simulink model "ext_mode_intro"  (R2017b)
settings: Solver=FixedStepDiscrete  StartTime=0.0  StopTime=inf  FixedStep=1/100  RelTol=1e-3  EnableMultiTasking=on
InitFcn:
  | GainTune = 1;
  | alignTime = floor(398.001 * Ts);
  | EAS2TAS = 1;
  | LatDegInit = 1;
  | LngDegInit = 1;
  | msecVelDelay = 300;
  | msecPosDelay = 300;
  | msecHgtDelay = 420;
  | msecMagDelay = 30;
  | msecTasDelay = 200;
libraries: simulink x9, pixhawk_slib_sensors_actuators x3, simulink_need_slupdate x2
(part 2 of 4)

== matlab function ext_mode_intro/EKF/EKF/Subsystem/Predict Covariance ==
  data: deltaAngle input; deltaVelocity input; nextP output; states input; P input; dtIMU input; onGround input; useAirspeed input; useCompass input
%#codegen
function nextP  = CovariancePrediction(deltaAngle, ...
    deltaVelocity, ...
    states,...
    P, ...  % Previous state covariance matrix
    dtIMU, ... % IMU and prediction time step
    onGround, ... % Boolean to indicate when on ground
    useAirspeed, ... % Boolean to indicate that airspeed sensing is being used
    useCompass) % Boolean to indicate that a magnetometer is being used

dtCovPred = 0.0; % time between covariance prediction updates

persistent storedDelAng;
if isempty(storedDelAng)
    storedDelAng = single([0;0;0]);
end
persistent storedDelVel;
if isempty(storedDelVel)
    storedDelVel = single([0;0;0]);
end
persistent dt;
if isempty(dt)
    dt = single(0.0);
end
persistent skipCount;
if isempty(skipCount)
    skipCount = 0;
end

storedDelAng = storedDelAng + deltaAngle;
storedDelVel = storedDelVel + deltaVelocity;
dt = dt + dtIMU;

if dt >= dtCovPred
    
    % Set the filter process noise - this consists of a very small amount to
    % cover processing errors. IMU errors are already built into the
    % equations
    % It  includes the process noise required for evolution of the IMU bias
    % errors, wind velocity and magnetic field states
    
    windVelSigma  = single(dt*0.1); % 0.1 m/s/s
    dAngBiasSigma = single(dt*0.05/3600*pi/180);
    dVelBiasSigma = single(dt*0.01/60);
    magEarthSigma = single(dt*10/60); % 10 mgauss per minute
    magBodySigma  = single(dt*100/60); % 100 mgauss per minute - allow to adapt more rapidly due to changes in airframe
    
    processNoise = [1e-9*ones(1,10), dAngBiasSigma*[1 1 1], dVelBiasSigma*[1 1 1], windVelSigma*[1 1], magEarthSigma*[1 1 1], magBodySigma*[1 1 1]].^2;
    
    % Specify the estimated errors on the delta angles and delta velocities
    daxCov = (dt*25.0/60*pi/180)^2;
    dayCov = (dt*25.0/60*pi/180)^2;
    dazCov = (dt*25.0/60*pi/180)^2;
    dvxCov = (dt*0.5)^2;
    dvyCov = (dt*0.5)^2;
    dvzCov = (dt*0.5)^2;
    
    dvx = deltaVelocity(1);
    dvy = deltaVelocity(2);
    dvz = deltaVelocity(3);
    dax = deltaAngle(1);
    day = deltaAngle(2);
    daz = deltaAngle(3);
    
    q0 = states(1);
    q1 = states(2);
    q2 = states(3);
    q3 = states(4);
    
    vn = states(5);
    ve = states(6);
    vd = states(7);
    
    pn = states(8);
    pe = states(9);
    pd = states(10);
    
    dax_b = states(11);
    day_b = states(12);
    daz_b = states(13);
    
    dvx_b = states(14);
    dvy_b = states(15);
    dvz_b = states(16);
    
    vwn = states(17);
    vwe = states(18);
    
    magN = states(19);
    magE = states(20);
    magD = states(21);
    
    magX = states(22);
    magY = states(23);
    magZ = states(24);
    
    % Predicted covariance
    
    SF = single(zeros(21,1));
    SF(1) = dvz - dvz_b;
    SF(2) = dvy - dvy_b;
    SF(3) = dvx - dvx_b;
    SF(4) = 2*q1*SF(3) + 2*q2*SF(2) + 2*q3*SF(1);
    SF(5) = 2*q0*SF(2) - 2*q1*SF(1) + 2*q3*SF(3);
    SF(6) = 2*q0*SF(3) + 2*q2*SF(1) - 2*q3*SF(2);
    SF(7) = day/2 - day_b/2;
    SF(8) = daz/2 - daz_b/2;
    SF(9) = dax/2 - dax_b/2;
    SF(10) = dax_b/2 - dax/2;
    SF(11) = daz_b/2 - daz/2;
    SF(12) = day_b/2 - day/2;
    SF(13) = 2*q1*SF(2);
    SF(14) = 2*q0*SF(1);
    SF(15) = q1/2;
    SF(16) = q2/2;
    SF(17) = q3/2;
    SF(18) = q3^2;
    SF(19) = q2^2;
    SF(20) = q1^2;
    SF(21) = q0^2;
    
    SG = single(zeros(8,1));
    SG(1) = q0/2;
    SG(2) = q3^2;
    SG(3) = q2^2;
    SG(4) = q1^2;
    SG(5) = q0^2;
    SG(6) = 2*q2*q3;
    SG(7) = 2*q1*q3;
    SG(8) = 2*q1*q2;
    
    SQ = single(zeros(11,1));
    SQ(1) = dvzCov*(SG(6) - 2*q0*q1)*(SG(2) - SG(3) - SG(4) + SG(5)) - dvyCov*(SG(6) + 2*q0*q1)*(SG(2) - SG(3) + SG(4) - SG(5)) + dvxCov*(SG(7) - 2*q0*q2)*(SG(8) + 2*q0*q3);
    SQ(2) = dvzCov*(SG(7) + 2*q0*q2)*(SG(2) - SG(3) - SG(4) + SG(5)) - dvxCov*(SG(7) - 2*q0*q2)*(SG(2) + SG(3) - SG(4) - SG(5)) + dvyCov*(SG(6) + 2*q0*q1)*(SG(8) - 2*q0*q3);
    SQ(3) = dvzCov*(SG(6) - 2*q0*q1)*(SG(7) + 2*q0*q2) - dvyCov*(SG(8) - 2*q0*q3)*(SG(2) - SG(3) + SG(4) - SG(5)) - dvxCov*(SG(8) + 2*q0*q3)*(SG(2) + SG(3) - SG(4) - SG(5));
    SQ(4) = (dayCov*q1*SG(1))/2 - (dazCov*q1*SG(1))/2 - (daxCov*q2*q3)/4;
    SQ(5) = (dazCov*q2*SG(1))/2 - (daxCov*q2*SG(1))/2 - (dayCov*q1*q3)/4;
    SQ(6) = (daxCov*q3*SG(1))/2 - (dayCov*q3*SG(1))/2 - (dazCov*q1*q2)/4;
    SQ(7) = (daxCov*q1*q2)/4 - (dazCov*q3*SG(1))/2 - (dayCov*q1*q2)/4;
    SQ(8) = (dazCov*q1*q3)/4 - (daxCov*q1*q3)/4 - (dayCov*q2*SG(1))/2;
    SQ(9) = (dayCov*q2*q3)/4 - (daxCov*q1*SG(1))/2 - (dazCov*q2*q3)/4;
    SQ(10) = SG(1)^2;
    SQ(11) = q1^2;
    
    SPP = single(zeros(13,1));
    SPP(1) = SF(13) + SF(14) - 2*q2*SF(3);
    SPP(2) = SF(18) - SF(19) - SF(20) + SF(21);
    SPP(3) = SF(18) - SF(19) + SF(20) - SF(21);
    SPP(4) = SF(18) + SF(19) - SF(20) - SF(21);
    SPP(5) = 2*q0*SF(3) + 2*q2*SF(1) - 2*q3*SF(2);
    SPP(6) = 2*q0*SF(2) - 2*q1*SF(1) + 2*q3*SF(3);
    SPP(7) = 2*q0*q2 - 2*q1*q3;
    SPP(8) = 2*q0*q1 - 2*q2*q3;
    SPP(9) = 2*q0*q3 - 2*q1*q2;
    SPP(10) = 2*q0*q1 + 2*q2*q3;
    SPP(11) = 2*q0*q3 + 2*q1*q2;
    SPP(12) = 2*q0*q2 + 2*q1*q3;
    SPP(13) = SF(17);
    
    nextP = single(zeros(24,24));
    nextP(1,1) = P(1,1) + P(2,1)*SF(10) + P(3,1)*SF(12) + P(4,1)*SF(11) + P(11,1)*SF(15) + P(12,1)*SF(16) + P(13,1)*SPP(13) + (daxCov*SQ(11))/4 + SF(10)*(P(1,2) + P(2,2)*SF(10) + P(3,2)*SF(12) + P(4,2)*SF(11) + P(11,2)*SF(15) + P(12,2)*SF(16) + P(13,2)*SPP(13)) + SF(12)*(P(1,3) + P(2,3)*SF(10) + P(3,3)*SF(12) + P(4,3)*SF(11) + P(11,3)*SF(15) + P(12,3)*SF(16) + P(13,3)*SPP(13)) + SF(11)*(P(1,4) + P(2,4)*SF(10) + P(3,4)*SF(12) + P(4,4)*SF(11) + P(11,4)*SF(15) + P(12,4)*SF(16) + P(13,4)*SPP(13)) + SF(15)*(P(1,11) + P(2,11)*SF(10) + P(3,11)*SF(12) + P(4,11)*SF(11) + P(11,11)*SF(15) + P(12,11)*SF(16) + P(13,11)*SPP(13)) + SF(16)*(P(1,12) + P(2,12)*SF(10) + P(3,12)*SF(12) + P(4,12)*SF(11) + P(11,12)*SF(15) + P(12,12)*SF(16) + P(13,12)*SPP(13)) + SPP(13)*(P(1,13) + P(2,13)*SF(10) + P(3,13)*SF(12) + P(4,13)*SF(11) + P(11,13)*SF(15) + P(12,13)*SF(16) + P(13,13)*SPP(13)) + (dayCov*q2^2)/4 + (dazCov*q3^2)/4;
    nextP(1,2) = P(1,2) + SQ(9) + P(2,2)*SF(10) + P(3,2)*SF(12) + P(4,2)*SF(11) + P(11,2)*SF(15) + P(12,2)*SF(16) + P(13,2)*SPP(13) + SF(9)*(P(1,1) + P(2,1)*SF(10) + P(3,1)*SF(12) + P(4,1)*SF(11) + P(11,1)*SF(15) + P(12,1)*SF(16) + P(13,1)*SPP(13)) + SF(8)*(P(1,3) + P(2,3)*SF(10) + P(3,3)*SF(12) + P(4,3)*SF(11) + P(11,3)*SF(15) + P(12,3)*SF(16) + P(13,3)*SPP(13)) + SF(12)*(P(1,4) + P(2,4)*SF(10) + P(3,4)*SF(12) + P(4,4)*SF(11) + P(11,4)*SF(15) + P(12,4)*SF(16) + P(13,4)*SPP(13)) - SF(16)*(P(1,13) + P(2,13)*SF(10) + P(3,13)*SF(12) + P(4,13)*SF(11) + P(11,13)*SF(15) + P(12,13)*SF(16) + P(13,13)*SPP(13)) + SPP(13)*(P(1,12) + P(2,12)*SF(10) + P(3,12)*SF(12) + P(4,12)*SF(11) + P(11,12)*SF(15) + P(12,12)*SF(16) + P(13,12)*SPP(13)) - (q0*(P(1,11) + P(2,11)*SF(10) + P(3,11)*SF(12) + P(4,11)*SF(11) + P(11,11)*SF(15) + P(12,11)*SF(16) + P(13,11)*SPP(13)))/2;
    nextP(1,3) = P(1,3) + SQ(8) + P(2,3)*SF(10) + P(3,3)*SF(12) + P(4,3)*SF(11) + P(11,3)*SF(15) + P(12,3)*SF(16) + P(13,3)*SPP(13) + SF(7)*(P(1,1) + P(2,1)*SF(10) + P(3,1)*SF(12) + P(4,1)*SF(11) + P(11,1)*SF(15) + P(12,1)*SF(16) + P(13,1)*SPP(13)) + SF(11)*(P(1,2) + P(2,2)*SF(10) + P(3,2)*SF(12) + P(4,2)*SF(11) + P(11,2)*SF(15) + P(12,2)*SF(16) + P(13,2)*SPP(13)) + SF(9)*(P(1,4) + P(2,4)*SF(10) + P(3,4)*SF(12) + P(4,4)*SF(11) + P(11,4)*SF(15) + P(12,4)*SF(16) + P(13,4)*SPP(13)) + SF(15)*(P(1,13) + P(2,13)*SF(10) + P(3,13)*SF(12) + P(4,13)*SF(11) + P(11,13)*SF(15) + P(12,13)*SF(16) + P(13,13)*SPP(13)) - SPP(13)*(P(1,11) + P(2,11)*SF(10) + P(3,11)*SF(12) + P(4,11)*SF(11) + P(11,11)*SF(15) + P(12,11)*SF(16) + P(13,11)*SPP(13)) - (q0*(P(1,12) + P(2,12)*SF(10) + P(3,12)*SF(12) + P(4,12)*SF(11) + P(11,12)*SF(15) + P(12,12)*SF(16) + P(13,12)*SPP(13)))/2;
    nextP(1,4) = P(1,4) + SQ(7) + P(2,4)*SF(10) + P(3,4)*SF(12) + P(4,4)*SF(11) + P(11,4)*SF(15) + P(12,4)*SF(16) + P(13,4)*SPP(13) + SF(8)*(P(1,1) + P(2,1)*SF(10) + P(3,1)*SF(12) + P(4,1)*SF(11) + P(11,1)*SF(15) + P(12,1)*SF(16) + P(13,1)*SPP(13)) + SF(7)*(P(1,2) + P(2,2)*SF(10) + P(3,2)*SF(12) + P(4,2)*SF(11) + P(11,2)*SF(15) + P(12,2)*SF(16) + P(13,2)*SPP(13)) + SF(10)*(P(1,3) + P(2,3)*SF(10) + P(3,3)*SF(12) + P(4,3)*SF(11) + P(11,3)*SF(15) + P(12,3)*SF(16) + P(13,3)*SPP(13)) + SF(16)*(P(1,11) + P(2,11)*SF(10) + P(3,11)*SF(12) + P(4,11)*SF(11) + P(11,11)*SF(15) + P(12,11)*SF(16) + P(13,11)*SPP(13)) - SF(15)*(P(1,12) + P(2,12)*SF(10) + P(3,12)*SF(12) + P(4,12)*SF(11) + P(11,12)*SF(15) + P(12,12)*SF(16) + P(13,12)*SPP(13)) - (q0*(P(1,13) + P(2,13)*SF(10) + P(3,13)*SF(12) + P(4,13)*SF(11) + P(11,13)*SF(15) + P(12,13)*SF(16) + P(13,13)*SPP(13)))/2;
    nextP(1,5) = P(1,5) + P(2,5)*SF(10) + P(3,5)*SF(12) + P(4,5)*SF(11) + P(11,5)*SF(15) + P(12,5)*SF(16) + P(13,5)*SPP(13) + SF(6)*(P(1,1) + P(2,1)*SF(10) + P(3,1)*SF(12) + P(4,1)*SF(11) + P(11,1)*SF(15) + P(12,1)*SF(16) + P(13,1)*SPP(13)) + SF(4)*(P(1,2) + P(2,2)*SF(10) + P(3,2)*SF(12) + P(4,2)*SF(11) + P(11,2)*SF(15) + P(12,2)*SF(16) + P(13,2)*SPP(13)) + SPP(1)*(P(1,3) + P(2,3)*SF(10) + P(3,3)*SF(12) + P(4,3)*SF(11) + P(11,3)*SF(15) + P(12,3)*SF(16) + P(13,3)*SPP(13)) - SPP(6)*(P(1,4) + P(2,4)*SF(10) + P(3,4)*SF(12) + P(4,4)*SF(11) + P(11,4)*SF(15) + P(12,4)*SF(16) + P(13,4)*SPP(13)) + SPP(4)*(P(1,14) + P(2,14)*SF(10) + P(3,14)*SF(12) + P(4,14)*SF(11) + P(11,14)*SF(15) + P(12,14)*SF(16) + P(13,14)*SPP(13)) - SPP(12)*(P(1,16) + P(2,16)*SF(10) + P(3,16)*SF(12) + P(4,16)*SF(11) + P(11,16)*SF(15) + P(12,16)*SF(16) + P(13,16)*SPP(13)) + (2*q0*q3 - 2*q1*q2)*(P(1,15) + P(2,15)*SF(10) + P(3,15)*SF(12) + P(4,15)*SF(11) + P(11,15)*SF(15) + P(12,15)*SF(16) + P(13,15)*SPP(13));
    nextP(1,6) = P(1,6) + P(2,6)*SF(10) + P(3,6)*SF(12) + P(4,6)*SF(11) + P(11,6)*SF(15) + P(12,6)*SF(16) + P(13,6)*SPP(13) + SF(5)*(P(1,1) + P(2,1)*SF(10) + P(3,1)*SF(12) + P(4,1)*SF(11) + P(11,1)*SF(15) + P(12,1)*SF(16) + P(13,1)*SPP(13)) + SF(4)*(P(1,3) + P(2,3)*SF(10) + P(3,3)*SF(12) + P(4,3)*SF(11) + P(11,3)*SF(15) + P(12,3)*SF(16) + P(13,3)*SPP(13)) + SF(6)*(P(1,4) + P(2,4)*SF(10) + P(3,4)*SF(12) + P(4,4)*SF(11) + P(11,4)*SF(15) + P(12,4)*SF(16) + P(13,4)*SPP(13)) - SPP(1)*(P(1,2) + P(2,2)*SF(10) + P(3,2)*SF(12) + P(4,2)*SF(11) + P(11,2)*SF(15) + P(12,2)*SF(16) + P(13,2)*SPP(13)) + SPP(3)*(P(1,15) + P(2,15)*SF(10) + P(3,15)*SF(12) + P(4,15)*SF(11) + P(11,15)*SF(15) + P(12,15)*SF(16) + P(13,15)*SPP(13)) - SPP(11)*(P(1,14) + P(2,14)*SF(10) + P(3,14)*SF(12) + P(4,14)*SF(11) + P(11,14)*SF(15) + P(12,14)*SF(16) + P(13,14)*SPP(13)) + (2*q0*q1 - 2*q2*q3)*(P(1,16) + P(2,16)*SF(10) + P(3,16)*SF(12) + P(4,16)*SF(11) + P(11,16)*SF(15) + P(12,16)*SF(16) + P(13,16)*SPP(13));
    nextP(1,7) = P(1,7) + P(2,7)*SF(10) + P(3,7)*SF(12) + P(4,7)*SF(11) + P(11,7)*SF(15) + P(12,7)*SF(16) + P(13,7)*SPP(13) + SF(5)*(P(1,2) + P(2,2)*SF(10) + P(3,2)*SF(12) + P(4,2)*SF(11) + P(11,2)*SF(15) + P(12,2)*SF(16) + P(13,2)*SPP(13)) + SF(4)*(P(1,4) + P(2,4)*SF(10) + P(3,4)*SF(12) + P(4,4)*SF(11) + P(11,4)*SF(15) + P(12,4)*SF(16) + P(13,4)*SPP(13)) + SPP(1)*(P(1,1) + P(2,1)*SF(10) + P(3,1)*SF(12) + P(4,1)*SF(11) + P(11,1)*SF(15) + P(12,1)*SF(16) + P(13,1)*SPP(13)) - SPP(5)*(P(1,3) + P(2,3)*SF(10) + P(3,3)*SF(12) + P(4,3)*SF(11) + P(11,3)*SF(15) + P(12,3)*SF(16) + P(13,3)*SPP(13)) + SPP(7)*(P(1,14) + P(2,14)*SF(10) + P(3,14)*SF(12) + P(4,14)*SF(11) + P(11,14)*SF(15) + P(12,14)*SF(16) + P(13,14)*SPP(13)) - SPP(2)*(P(1,16) + P(2,16)*SF(10) + P(3,16)*SF(12) + P(4,16)*SF(11) + P(11,16)*SF(15) + P(12,16)*SF(16) + P(13,16)*SPP(13)) - SPP(10)*(P(1,15) + P(2,15)*SF(10) + P(3,15)*SF(12) + P(4,15)*SF(11) + P(11,15)*SF(15) + P(12,15)*SF(16) + P(13,15)*SPP(13));
    nextP(1,8) = P(1,8) + P(2,8)*SF(10) + P(3,8)*SF(12) + P(4,8)*SF(11) + P(11,8)*SF(15) + P(12,8)*SF(16) + P(13,8)*SPP(13) + dt*(P(1,5) + P(2,5)*SF(10) + P(3,5)*SF(12) + P(4,5)*SF(11) + P(11,5)*SF(15) + P(12,5)*SF(16) + P(13,5)*SPP(13));
    nextP(1,9) = P(1,9) + P(2,9)*SF(10) + P(3,9)*SF(12) + P(4,9)*SF(11) + P(11,9)*SF(15) + P(12,9)*SF(16) + P(13,9)*SPP(13) + dt*(P(1,6) + P(2,6)*SF(10) + P(3,6)*SF(12) + P(4,6)*SF(11) + P(11,6)*SF(15) + P(12,6)*SF(16) + P(13,6)*SPP(13));
    nextP(1,10) = P(1,10) + P(2,10)*SF(10) + P(3,10)*SF(12) + P(4,10)*SF(11) + P(11,10)*SF(15) + P(12,10)*SF(16) + P(13,10)*SPP(13) + dt*(P(1,7) + P(2,7)*SF(10) + P(3,7)*SF(12) + P(4,7)*SF(11) + P(11,7)*SF(15) + P(12,7)*SF(16) + P(13,7)*SPP(13));
    nextP(1,11) = P(1,11) + P(2,11)*SF(10) + P(3,11)*SF(12) + P(4,11)*SF(11) + P(11,11)*SF(15) + P(12,11)*SF(16) + P(13,11)*SPP(13);
    nextP(1,12) = P(1,12) + P(2,12)*SF(10) + P(3,12)*SF(12) + P(4,12)*SF(11) + P(11,12)*SF(15) + P(12,12)*SF(16) + P(13,12)*SPP(13);
    nextP(1,13) = P(1,13) + P(2,13)*SF(10) + P(3,13)*SF(12) + P(4,13)*SF(11) + P(11,13)*SF(15) + P(12,13)*SF(16) + P(13,13)*SPP(13);
    nextP(1,14) = P(1,14) + P(2,14)*SF(10) + P(3,14)*SF(12) + P(4,14)*SF(11) + P(11,14)*SF(15) + P(12,14)*SF(16) + P(13,14)*SPP(13);
    nextP(1,15) = P(1,15) + P(2,15)*SF(10) + P(3,15)*SF(12) + P(4,15)*SF(11) + P(11,15)*SF(15) + P(12,15)*SF(16) + P(13,15)*SPP(13);
    nextP(1,16) = P(1,16) + P(2,16)*SF(10) + P(3,16)*SF(12) + P(4,16)*SF(11) + P(11,16)*SF(15) + P(12,16)*SF(16) + P(13,16)*SPP(13);
    nextP(1,17) = P(1,17) + P(2,17)*SF(10) + P(3,17)*SF(12) + P(4,17)*SF(11) + P(11,17)*SF(15) + P(12,17)*SF(16) + P(13,17)*SPP(13);
    nextP(1,18) = P(1,18) + P(2,18)*SF(10) + P(3,18)*SF(12) + P(4,18)*SF(11) + P(11,18)*SF(15) + P(12,18)*SF(16) + P(13,18)*SPP(13);
    nextP(1,19) = P(1,19) + P(2,19)*SF(10) + P(3,19)*SF(12) + P(4,19)*SF(11) + P(11,19)*SF(15) + P(12,19)*SF(16) + P(13,19)*SPP(13);
    nextP(1,20) = P(1,20) + P(2,20)*SF(10) + P(3,20)*SF(12) + P(4,20)*SF(11) + P(11,20)*SF(15) + P(12,20)*SF(16) + P(13,20)*SPP(13);
    nextP(1,21) = P(1,21) + P(2,21)*SF(10) + P(3,21)*SF(12) + P(4,21)*SF(11) + P(11,21)*SF(15) + P(12,21)*SF(16) + P(13,21)*SPP(13);
    nextP(1,22) = P(1,22) + P(2,22)*SF(10) + P(3,22)*SF(12) + P(4,22)*SF(11) + P(11,22)*SF(15) + P(12,22)*SF(16) + P(13,22)*SPP(13);
    nextP(1,23) = P(1,23) + P(2,23)*SF(10) + P(3,23)*SF(12) + P(4,23)*SF(11) + P(11,23)*SF(15) + P(12,23)*SF(16) + P(13,23)*SPP(13);
    nextP(1,24) = P(1,24) + P(2,24)*SF(10) + P(3,24)*SF(12) + P(4,24)*SF(11) + P(11,24)*SF(15) + P(12,24)*SF(16) + P(13,24)*SPP(13);
    nextP(2,1) = P(2,1) + SQ(9) + P(1,1)*SF(9) + P(3,1)*SF(8) + P(4,1)*SF(12) - P(13,1)*SF(16) + P(12,1)*SPP(13) - (P(11,1)*q0)/2 + SF(10)*(P(2,2) + P(1,2)*SF(9) + P(3,2)*SF(8) + P(4,2)*SF(12) - P(13,2)*SF(16) + P(12,2)*SPP(13) - (P(11,2)*q0)/2) + SF(12)*(P(2,3) + P(1,3)*SF(9) + P(3,3)*SF(8) + P(4,3)*SF(12) - P(13,3)*SF(16) + P(12,3)*SPP(13) - (P(11,3)*q0)/2) + SF(11)*(P(2,4) + P(1,4)*SF(9) + P(3,4)*SF(8) + P(4,4)*SF(12) - P(13,4)*SF(16) + P(12,4)*SPP(13) - (P(11,4)*q0)/2) + SF(15)*(P(2,11) + P(1,11)*SF(9) + P(3,11)*SF(8) + P(4,11)*SF(12) - P(13,11)*SF(16) + P(12,11)*SPP(13) - (P(11,11)*q0)/2) + SF(16)*(P(2,12) + P(1,12)*SF(9) + P(3,12)*SF(8) + P(4,12)*SF(12) - P(13,12)*SF(16) + P(12,12)*SPP(13) - (P(11,12)*q0)/2) + SPP(13)*(P(2,13) + P(1,13)*SF(9) + P(3,13)*SF(8) + P(4,13)*SF(12) - P(13,13)*SF(16) + P(12,13)*SPP(13) - (P(11,13)*q0)/2);
    nextP(2,2) = P(2,2) + P(1,2)*SF(9) + P(3,2)*SF(8) + P(4,2)*SF(12) - P(13,2)*SF(16) + P(12,2)*SPP(13) + daxCov*SQ(10) - (P(11,2)*q0)/2 + SF(9)*(P(2,1) + P(1,1)*SF(9) + P(3,1)*SF(8) + P(4,1)*SF(12) - P(13,1)*SF(16) + P(12,1)*SPP(13) - (P(11,1)*q0)/2) + SF(8)*(P(2,3) + P(1,3)*SF(9) + P(3,3)*SF(8) + P(4,3)*SF(12) - P(13,3)*SF(16) + P(12,3)*SPP(13) - (P(11,3)*q0)/2) + SF(12)*(P(2,4) + P(1,4)*SF(9) + P(3,4)*SF(8) + P(4,4)*SF(12) - P(13,4)*SF(16) + P(12,4)*SPP(13) - (P(11,4)*q0)/2) - SF(16)*(P(2,13) + P(1,13)*SF(9) + P(3,13)*SF(8) + P(4,13)*SF(12) - P(13,13)*SF(16) + P(12,13)*SPP(13) - (P(11,13)*q0)/2) + SPP(13)*(P(2,12) + P(1,12)*SF(9) + P(3,12)*SF(8) + P(4,12)*SF(12) - P(13,12)*SF(16) + P(12,12)*SPP(13) - (P(11,12)*q0)/2) + (dayCov*q3^2)/4 + (dazCov*q2^2)/4 - (q0*(P(2,11) + P(1,11)*SF(9) + P(3,11)*SF(8) + P(4,11)*SF(12) - P(13,11)*SF(16) + P(12,11)*SPP(13) - (P(11,11)*q0)/2))/2;
    nextP(2,3) = P(2,3) + SQ(6) + P(1,3)*SF(9) + P(3,3)*SF(8) + P(4,3)*SF(12) - P(13,3)*SF(16) + P(12,3)*SPP(13) - (P(11,3)*q0)/2 + SF(7)*(P(2,1) + P(1,1)*SF(9) + P(3,1)*SF(8) + P(4,1)*SF(12) - P(13,1)*SF(16) + P(12,1)*SPP(13) - (P(11,1)*q0)/2) + SF(11)*(P(2,2) + P(1,2)*SF(9) + P(3,2)*SF(8) + P(4,2)*SF(12) - P(13,2)*SF(16) + P(12,2)*SPP(13) - (P(11,2)*q0)/2) + SF(9)*(P(2,4) + P(1,4)*SF(9) + P(3,4)*SF(8) + P(4,4)*SF(12) - P(13,4)*SF(16) + P(12,4)*SPP(13) - (P(11,4)*q0)/2) + SF(15)*(P(2,13) + P(1,13)*SF(9) + P(3,13)*SF(8) + P(4,13)*SF(12) - P(13,13)*SF(16) + P(12,13)*SPP(13) - (P(11,13)*q0)/2) - SPP(13)*(P(2,11) + P(1,11)*SF(9) + P(3,11)*SF(8) + P(4,11)*SF(12) - P(13,11)*SF(16) + P(12,11)*SPP(13) - (P(11,11)*q0)/2) - (q0*(P(2,12) + P(1,12)*SF(9) + P(3,12)*SF(8) + P(4,12)*SF(12) - P(13,12)*SF(16) + P(12,12)*SPP(13) - (P(11,12)*q0)/2))/2;
    nextP(2,4) = P(2,4) + SQ(5) + P(1,4)*SF(9) + P(3,4)*SF(8) + P(4,4)*SF(12) - P(13,4)*SF(16) + P(12,4)*SPP(13) - (P(11,4)*q0)/2 + SF(8)*(P(2,1) + P(1,1)*SF(9) + P(3,1)*SF(8) + P(4,1)*SF(12) - P(13,1)*SF(16) + P(12,1)*SPP(13) - (P(11,1)*q0)/2) + SF(7)*(P(2,2) + P(1,2)*SF(9) + P(3,2)*SF(8) + P(4,2)*SF(12) - P(13,2)*SF(16) + P(12,2)*SPP(13) - (P(11,2)*q0)/2) + SF(10)*(P(2,3) + P(1,3)*SF(9) + P(3,3)*SF(8) + P(4,3)*SF(12) - P(13,3)*SF(16) + P(12,3)*SPP(13) - (P(11,3)*q0)/2) + SF(16)*(P(2,11) + P(1,11)*SF(9) + P(3,11)*SF(8) + P(4,11)*SF(12) - P(13,11)*SF(16) + P(12,11)*SPP(13) - (P(11,11)*q0)/2) - SF(15)*(P(2,12) + P(1,12)*SF(9) + P(3,12)*SF(8) + P(4,12)*SF(12) - P(13,12)*SF(16) + P(12,12)*SPP(13) - (P(11,12)*q0)/2) - (q0*(P(2,13) + P(1,13)*SF(9) + P(3,13)*SF(8) + P(4,13)*SF(12) - P(13,13)*SF(16) + P(12,13)*SPP(13) - (P(11,13)*q0)/2))/2;
    nextP(2,5) = P(2,5) + P(1,5)*SF(9) + P(3,5)*SF(8) + P(4,5)*SF(12) - P(13,5)*SF(16) + P(12,5)*SPP(13) - (P(11,5)*q0)/2 + SF(6)*(P(2,1) + P(1,1)*SF(9) + P(3,1)*SF(8) + P(4,1)*SF(12) - P(13,1)*SF(16) + P(12,1)*SPP(13) - (P(11,1)*q0)/2) + SF(4)*(P(2,2) + P(1,2)*SF(9) + P(3,2)*SF(8) + P(4,2)*SF(12) - P(13,2)*SF(16) + P(12,2)*SPP(13) - (P(11,2)*q0)/2) + SPP(1)*(P(2,3) + P(1,3)*SF(9) + P(3,3)*SF(8) + P(4,3)*SF(12) - P(13,3)*SF(16) + P(12,3)*SPP(13) - (P(11,3)*q0)/2) - SPP(6)*(P(2,4) + P(1,4)*SF(9) + P(3,4)*SF(8) + P(4,4)*SF(12) - P(13,4)*SF(16) + P(12,4)*SPP(13) - (P(11,4)*q0)/2) + SPP(4)*(P(2,14) + P(1,14)*SF(9) + P(3,14)*SF(8) + P(4,14)*SF(12) - P(13,14)*SF(16) + P(12,14)*SPP(13) - (P(11,14)*q0)/2) + SPP(9)*(P(2,15) + P(1,15)*SF(9) + P(3,15)*SF(8) + P(4,15)*SF(12) - P(13,15)*SF(16) + P(12,15)*SPP(13) - (P(11,15)*q0)/2) - SPP(12)*(P(2,16) + P(1,16)*SF(9) + P(3,16)*SF(8) + P(4,16)*SF(12) - P(13,16)*SF(16) + P(12,16)*SPP(13) - (P(11,16)*q0)/2);
    nextP(2,6) = P(2,6) + P(1,6)*SF(9) + P(3,6)*SF(8) + P(4,6)*SF(12) - P(13,6)*SF(16) + P(12,6)*SPP(13) - (P(11,6)*q0)/2 + SF(5)*(P(2,1) + P(1,1)*SF(9) + P(3,1)*SF(8) + P(4,1)*SF(12) - P(13,1)*SF(16) + P(12,1)*SPP(13) - (P(11,1)*q0)/2) + SF(4)*(P(2,3) + P(1,3)*SF(9) + P(3,3)*SF(8) + P(4,3)*SF(12) - P(13,3)*SF(16) + P(12,3)*SPP(13) - (P(11,3)*q0)/2) + SF(6)*(P(2,4) + P(1,4)*SF(9) + P(3,4)*SF(8) + P(4,4)*SF(12) - P(13,4)*SF(16) + P(12,4)*SPP(13) - (P(11,4)*q0)/2) - SPP(1)*(P(2,2) + P(1,2)*SF(9) + P(3,2)*SF(8) + P(4,2)*SF(12) - P(13,2)*SF(16) + P(12,2)*SPP(13) - (P(11,2)*q0)/2) + SPP(3)*(P(2,15) + P(1,15)*SF(9) + P(3,15)*SF(8) + P(4,15)*SF(12) - P(13,15)*SF(16) + P(12,15)*SPP(13) - (P(11,15)*q0)/2) - SPP(11)*(P(2,14) + P(1,14)*SF(9) + P(3,14)*SF(8) + P(4,14)*SF(12) - P(13,14)*SF(16) + P(12,14)*SPP(13) - (P(11,14)*q0)/2) + SPP(8)*(P(2,16) + P(1,16)*SF(9) + P(3,16)*SF(8) + P(4,16)*SF(12) - P(13,16)*SF(16) + P(12,16)*SPP(13) - (P(11,16)*q0)/2);
    nextP(2,7) = P(2,7) + P(1,7)*SF(9) + P(3,7)*SF(8) + P(4,7)*SF(12) - P(13,7)*SF(16) + P(12,7)*SPP(13) - (P(11,7)*q0)/2 + SF(5)*(P(2,2) + P(1,2)*SF(9) + P(3,2)*SF(8) + P(4,2)*SF(12) - P(13,2)*SF(16) + P(12,2)*SPP(13) - (P(11,2)*q0)/2) + SF(4)*(P(2,4) + P(1,4)*SF(9) + P(3,4)*SF(8) + P(4,4)*SF(12) - P(13,4)*SF(16) + P(12,4)*SPP(13) - (P(11,4)*q0)/2) + SPP(1)*(P(2,1) + P(1,1)*SF(9) + P(3,1)*SF(8) + P(4,1)*SF(12) - P(13,1)*SF(16) + P(12,1)*SPP(13) - (P(11,1)*q0)/2) - SPP(5)*(P(2,3) + P(1,3)*SF(9) + P(3,3)*SF(8) + P(4,3)*SF(12) - P(13,3)*SF(16) + P(12,3)*SPP(13) - (P(11,3)*q0)/2) + SPP(7)*(P(2,14) + P(1,14)*SF(9) + P(3,14)*SF(8) + P(4,14)*SF(12) - P(13,14)*SF(16) + P(12,14)*SPP(13) - (P(11,14)*q0)/2) - SPP(2)*(P(2,16) + P(1,16)*SF(9) + P(3,16)*SF(8) + P(4,16)*SF(12) - P(13,16)*SF(16) + P(12,16)*SPP(13) - (P(11,16)*q0)/2) - SPP(10)*(P(2,15) + P(1,15)*SF(9) + P(3,15)*SF(8) + P(4,15)*SF(12) - P(13,15)*SF(16) + P(12,15)*SPP(13) - (P(11,15)*q0)/2);
    nextP(2,8) = P(2,8) + P(1,8)*SF(9) + P(3,8)*SF(8) + P(4,8)*SF(12) - P(13,8)*SF(16) + P(12,8)*SPP(13) - (P(11,8)*q0)/2 + dt*(P(2,5) + P(1,5)*SF(9) + P(3,5)*SF(8) + P(4,5)*SF(12) - P(13,5)*SF(16) + P(12,5)*SPP(13) - (P(11,5)*q0)/2);
    nextP(2,9) = P(2,9) + P(1,9)*SF(9) + P(3,9)*SF(8) + P(4,9)*SF(12) - P(13,9)*SF(16) + P(12,9)*SPP(13) - (P(11,9)*q0)/2 + dt*(P(2,6) + P(1,6)*SF(9) + P(3,6)*SF(8) + P(4,6)*SF(12) - P(13,6)*SF(16) + P(12,6)*SPP(13) - (P(11,6)*q0)/2);
    nextP(2,10) = P(2,10) + P(1,10)*SF(9) + P(3,10)*SF(8) + P(4,10)*SF(12) - P(13,10)*SF(16) + P(12,10)*SPP(13) - (P(11,10)*q0)/2 + dt*(P(2,7) + P(1,7)*SF(9) + P(3,7)*SF(8) + P(4,7)*SF(12) - P(13,7)*SF(16) + P(12,7)*SPP(13) - (P(11,7)*q0)/2);
    nextP(2,11) = P(2,11) + P(1,11)*SF(9) + P(3,11)*SF(8) + P(4,11)*SF(12) - P(13,11)*SF(16) + P(12,11)*SPP(13) - (P(11,11)*q0)/2;
    nextP(2,12) = P(2,12) + P(1,12)*SF(9) + P(3,12)*SF(8) + P(4,12)*SF(12) - P(13,12)*SF(16) + P(12,12)*SPP(13) - (P(11,12)*q0)/2;
    nextP(2,13) = P(2,13) + P(1,13)*SF(9) + P(3,13)*SF(8) + P(4,13)*SF(12) - P(13,13)*SF(16) + P(12,13)*SPP(13) - (P(11,13)*q0)/2;
    nextP(2,14) = P(2,14) + P(1,14)*SF(9) + P(3,14)*SF(8) + P(4,14)*SF(12) - P(13,14)*SF(16) + P(12,14)*SPP(13) - (P(11,14)*q0)/2;
    nextP(2,15) = P(2,15) + P(1,15)*SF(9) + P(3,15)*SF(8) + P(4,15)*SF(12) - P(13,15)*SF(16) + P(12,15)*SPP(13) - (P(11,15)*q0)/2;
    nextP(2,16) = P(2,16) + P(1,16)*SF(9) + P(3,16)*SF(8) + P(4,16)*SF(12) - P(13,16)*SF(16) + P(12,16)*SPP(13) - (P(11,16)*q0)/2;
    nextP(2,17) = P(2,17) + P(1,17)*SF(9) + P(3,17)*SF(8) + P(4,17)*SF(12) - P(13,17)*SF(16) + P(12,17)*SPP(13) - (P(11,17)*q0)/2;
    nextP(2,18) = P(2,18) + P(1,18)*SF(9) + P(3,18)*SF(8) + P(4,18)*SF(12) - P(13,18)*SF(16) + P(12,18)*SPP(13) - (P(11,18)*q0)/2;
    nextP(2,19) = P(2,19) + P(1,19)*SF(9) + P(3,19)*SF(8) + P(4,19)*SF(12) - P(13,19)*SF(16) + P(12,19)*SPP(13) - (P(11,19)*q0)/2;
    nextP(2,20) = P(2,20) + P(1,20)*SF(9) + P(3,20)*SF(8) + P(4,20)*SF(12) - P(13,20)*SF(16) + P(12,20)*SPP(13) - (P(11,20)*q0)/2;
    nextP(2,21) = P(2,21) + P(1,21)*SF(9) + P(3,21)*SF(8) + P(4,21)*SF(12) - P(13,21)*SF(16) + P(12,21)*SPP(13) - (P(11,21)*q0)/2;
    nextP(2,22) = P(2,22) + P(1,22)*SF(9) + P(3,22)*SF(8) + P(4,22)*SF(12) - P(13,22)*SF(16) + P(12,22)*SPP(13) - (P(11,22)*q0)/2;
    nextP(2,23) = P(2,23) + P(1,23)*SF(9) + P(3,23)*SF(8) + P(4,23)*SF(12) - P(13,23)*SF(16) + P(12,23)*SPP(13) - (P(11,23)*q0)/2;
    nextP(2,24) = P(2,24) + P(1,24)*SF(9) + P(3,24)*SF(8) + P(4,24)*SF(12) - P(13,24)*SF(16) + P(12,24)*SPP(13) - (P(11,24)*q0)/2;
    nextP(3,1) = P(3,1) + SQ(8) + P(1,1)*SF(7) + P(2,1)*SF(11) + P(4,1)*SF(9) + P(13,1)*SF(15) - P(11,1)*SPP(13) - (P(12,1)*q0)/2 + SF(10)*(P(3,2) + P(1,2)*SF(7) + P(2,2)*SF(11) + P(4,2)*SF(9) + P(13,2)*SF(15) - P(11,2)*SPP(13) - (P(12,2)*q0)/2) + SF(12)*(P(3,3) + P(1,3)*SF(7) + P(2,3)*SF(11) + P(4,3)*SF(9) + P(13,3)*SF(15) - P(11,3)*SPP(13) - (P(12,3)*q0)/2) + SF(11)*(P(3,4) + P(1,4)*SF(7) + P(2,4)*SF(11) + P(4,4)*SF(9) + P(13,4)*SF(15) - P(11,4)*SPP(13) - (P(12,4)*q0)/2) + SF(15)*(P(3,11) + P(1,11)*SF(7) + P(2,11)*SF(11) + P(4,11)*SF(9) + P(13,11)*SF(15) - P(11,11)*SPP(13) - (P(12,11)*q0)/2) + SF(16)*(P(3,12) + P(1,12)*SF(7) + P(2,12)*SF(11) + P(4,12)*SF(9) + P(13,12)*SF(15) - P(11,12)*SPP(13) - (P(12,12)*q0)/2) + SPP(13)*(P(3,13) + P(1,13)*SF(7) + P(2,13)*SF(11) + P(4,13)*SF(9) + P(13,13)*SF(15) - P(11,13)*SPP(13) - (P(12,13)*q0)/2);
    nextP(3,2) = P(3,2) + SQ(6) + P(1,2)*SF(7) + P(2,2)*SF(11) + P(4,2)*SF(9) + P(13,2)*SF(15) - P(11,2)*SPP(13) - (P(12,2)*q0)/2 + SF(9)*(P(3,1) + P(1,1)*SF(7) + P(2,1)*SF(11) + P(4,1)*SF(9) + P(13,1)*SF(15) - P(11,1)*SPP(13) - (P(12,1)*q0)/2) + SF(8)*(P(3,3) + P(1,3)*SF(7) + P(2,3)*SF(11) + P(4,3)*SF(9) + P(13,3)*SF(15) - P(11,3)*SPP(13) - (P(12,3)*q0)/2) + SF(12)*(P(3,4) + P(1,4)*SF(7) + P(2,4)*SF(11) + P(4,4)*SF(9) + P(13,4)*SF(15) - P(11,4)*SPP(13) - (P(12,4)*q0)/2) - SF(16)*(P(3,13) + P(1,13)*SF(7) + P(2,13)*SF(11) + P(4,13)*SF(9) + P(13,13)*SF(15) - P(11,13)*SPP(13) - (P(12,13)*q0)/2) + SPP(13)*(P(3,12) + P(1,12)*SF(7) + P(2,12)*SF(11) + P(4,12)*SF(9) + P(13,12)*SF(15) - P(11,12)*SPP(13) - (P(12,12)*q0)/2) - (q0*(P(3,11) + P(1,11)*SF(7) + P(2,11)*SF(11) + P(4,11)*SF(9) + P(13,11)*SF(15) - P(11,11)*SPP(13) - (P(12,11)*q0)/2))/2;
    nextP(3,3) = P(3,3) + P(1,3)*SF(7) + P(2,3)*SF(11) + P(4,3)*SF(9) + P(13,3)*SF(15) - P(11,3)*SPP(13) + dayCov*SQ(10) + (dazCov*SQ(11))/4 - (P(12,3)*q0)/2 + SF(7)*(P(3,1) + P(1,1)*SF(7) + P(2,1)*SF(11) + P(4,1)*SF(9) + P(13,1)*SF(15) - P(11,1)*SPP(13) - (P(12,1)*q0)/2) + SF(11)*(P(3,2) + P(1,2)*SF(7) + P(2,2)*SF(11) + P(4,2)*SF(9) + P(13,2)*SF(15) - P(11,2)*SPP(13) - (P(12,2)*q0)/2) + SF(9)*(P(3,4) + P(1,4)*SF(7) + P(2,4)*SF(11) + P(4,4)*SF(9) + P(13,4)*SF(15) - P(11,4)*SPP(13) - (P(12,4)*q0)/2) + SF(15)*(P(3,13) + P(1,13)*SF(7) + P(2,13)*SF(11) + P(4,13)*SF(9) + P(13,13)*SF(15) - P(11,13)*SPP(13) - (P(12,13)*q0)/2) - SPP(13)*(P(3,11) + P(1,11)*SF(7) + P(2,11)*SF(11) + P(4,11)*SF(9) + P(13,11)*SF(15) - P(11,11)*SPP(13) - (P(12,11)*q0)/2) + (daxCov*q3^2)/4 - (q0*(P(3,12) + P(1,12)*SF(7) + P(2,12)*SF(11) + P(4,12)*SF(9) + P(13,12)*SF(15) - P(11,12)*SPP(13) - (P(12,12)*q0)/2))/2;
    nextP(3,4) = P(3,4) + SQ(4) + P(1,4)*SF(7) + P(2,4)*SF(11) + P(4,4)*SF(9) + P(13,4)*SF(15) - P(11,4)*SPP(13) - (P(12,4)*q0)/2 + SF(8)*(P(3,1) + P(1,1)*SF(7) + P(2,1)*SF(11) + P(4,1)*SF(9) + P(13,1)*SF(15) - P(11,1)*SPP(13) - (P(12,1)*q0)/2) + SF(7)*(P(3,2) + P(1,2)*SF(7) + P(2,2)*SF(11) + P(4,2)*SF(9) + P(13,2)*SF(15) - P(11,2)*SPP(13) - (P(12,2)*q0)/2) + SF(10)*(P(3,3) + P(1,3)*SF(7) + P(2,3)*SF(11) + P(4,3)*SF(9) + P(13,3)*SF(15) - P(11,3)*SPP(13) - (P(12,3)*q0)/2) + SF(16)*(P(3,11) + P(1,11)*SF(7) + P(2,11)*SF(11) + P(4,11)*SF(9) + P(13,11)*SF(15) - P(11,11)*SPP(13) - (P(12,11)*q0)/2) - SF(15)*(P(3,12) + P(1,12)*SF(7) + P(2,12)*SF(11) + P(4,12)*SF(9) + P(13,12)*SF(15) - P(11,12)*SPP(13) - (P(12,12)*q0)/2) - (q0*(P(3,13) + P(1,13)*SF(7) + P(2,13)*SF(11) + P(4,13)*SF(9) + P(13,13)*SF(15) - P(11,13)*SPP(13) - (P(12,13)*q0)/2))/2;
    nextP(3,5) = P(3,5) + P(1,5)*SF(7) + P(2,5)*SF(11) + P(4,5)*SF(9) + P(13,5)*SF(15) - P(11,5)*SPP(13) - (P(12,5)*q0)/2 + SF(6)*(P(3,1) + P(1,1)*SF(7) + P(2,1)*SF(11) + P(4,1)*SF(9) + P(13,1)*SF(15) - P(11,1)*SPP(13) - (P(12,1)*q0)/2) + SF(4)*(P(3,2) + P(1,2)*SF(7) + P(2,2)*SF(11) + P(4,2)*SF(9) + P(13,2)*SF(15) - P(11,2)*SPP(13) - (P(12,2)*q0)/2) + SPP(1)*(P(3,3) + P(1,3)*SF(7) + P(2,3)*SF(11) + P(4,3)*SF(9) + P(13,3)*SF(15) - P(11,3)*SPP(13) - (P(12,3)*q0)/2) - SPP(6)*(P(3,4) + P(1,4)*SF(7) + P(2,4)*SF(11) + P(4,4)*SF(9) + P(13,4)*SF(15) - P(11,4)*SPP(13) - (P(12,4)*q0)/2) + SPP(4)*(P(3,14) + P(1,14)*SF(7) + P(2,14)*SF(11) + P(4,14)*SF(9) + P(13,14)*SF(15) - P(11,14)*SPP(13) - (P(12,14)*q0)/2) + SPP(9)*(P(3,15) + P(1,15)*SF(7) + P(2,15)*SF(11) + P(4,15)*SF(9) + P(13,15)*SF(15) - P(11,15)*SPP(13) - (P(12,15)*q0)/2) - SPP(12)*(P(3,16) + P(1,16)*SF(7) + P(2,16)*SF(11) + P(4,16)*SF(9) + P(13,16)*SF(15) - P(11,16)*SPP(13) - (P(12,16)*q0)/2);
    nextP(3,6) = P(3,6) + P(1,6)*SF(7) + P(2,6)*SF(11) + P(4,6)*SF(9) + P(13,6)*SF(15) - P(11,6)*SPP(13) - (P(12,6)*q0)/2 + SF(5)*(P(3,1) + P(1,1)*SF(7) + P(2,1)*SF(11) + P(4,1)*SF(9) + P(13,1)*SF(15) - P(11,1)*SPP(13) - (P(12,1)*q0)/2) + SF(4)*(P(3,3) + P(1,3)*SF(7) + P(2,3)*SF(11) + P(4,3)*SF(9) + P(13,3)*SF(15) - P(11,3)*SPP(13) - (P(12,3)*q0)/2) + SF(6)*(P(3,4) + P(1,4)*SF(7) + P(2,4)*SF(11) + P(4,4)*SF(9) + P(13,4)*SF(15) - P(11,4)*SPP(13) - (P(12,4)*q0)/2) - SPP(1)*(P(3,2) + P(1,2)*SF(7) + P(2,2)*SF(11) + P(4,2)*SF(9) + P(13,2)*SF(15) - P(11,2)*SPP(13) - (P(12,2)*q0)/2) + SPP(3)*(P(3,15) + P(1,15)*SF(7) + P(2,15)*SF(11) + P(4,15)*SF(9) + P(13,15)*SF(15) - P(11,15)*SPP(13) - (P(12,15)*q0)/2) - SPP(11)*(P(3,14) + P(1,14)*SF(7) + P(2,14)*SF(11) + P(4,14)*SF(9) + P(13,14)*SF(15) - P(11,14)*SPP(13) - (P(12,14)*q0)/2) + SPP(8)*(P(3,16) + P(1,16)*SF(7) + P(2,16)*SF(11) + P(4,16)*SF(9) + P(13,16)*SF(15) - P(11,16)*SPP(13) - (P(12,16)*q0)/2);
    nextP(3,7) = P(3,7) + P(1,7)*SF(7) + P(2,7)*SF(11) + P(4,7)*SF(9) + P(13,7)*SF(15) - P(11,7)*SPP(13) - (P(12,7)*q0)/2 + SF(5)*(P(3,2) + P(1,2)*SF(7) + P(2,2)*SF(11) + P(4,2)*SF(9) + P(13,2)*SF(15) - P(11,2)*SPP(13) - (P(12,2)*q0)/2) + SF(4)*(P(3,4) + P(1,4)*SF(7) + P(2,4)*SF(11) + P(4,4)*SF(9) + P(13,4)*SF(15) - P(11,4)*SPP(13) - (P(12,4)*q0)/2) + SPP(1)*(P(3,1) + P(1,1)*SF(7) + P(2,1)*SF(11) + P(4,1)*SF(9) + P(13,1)*SF(15) - P(11,1)*SPP(13) - (P(12,1)*q0)/2) - SPP(5)*(P(3,3) + P(1,3)*SF(7) + P(2,3)*SF(11) + P(4,3)*SF(9) + P(13,3)*SF(15) - P(11,3)*SPP(13) - (P(12,3)*q0)/2) + SPP(7)*(P(3,14) + P(1,14)*SF(7) + P(2,14)*SF(11) + P(4,14)*SF(9) + P(13,14)*SF(15) - P(11,14)*SPP(13) - (P(12,14)*q0)/2) - SPP(2)*(P(3,16) + P(1,16)*SF(7) + P(2,16)*SF(11) + P(4,16)*SF(9) + P(13,16)*SF(15) - P(11,16)*SPP(13) - (P(12,16)*q0)/2) - SPP(10)*(P(3,15) + P(1,15)*SF(7) + P(2,15)*SF(11) + P(4,15)*SF(9) + P(13,15)*SF(15) - P(11,15)*SPP(13) - (P(12,15)*q0)/2);
    nextP(3,8) = P(3,8) + P(1,8)*SF(7) + P(2,8)*SF(11) + P(4,8)*SF(9) + P(13,8)*SF(15) - P(11,8)*SPP(13) - (P(12,8)*q0)/2 + dt*(P(3,5) + P(1,5)*SF(7) + P(2,5)*SF(11) + P(4,5)*SF(9) + P(13,5)*SF(15) - P(11,5)*SPP(13) - (P(12,5)*q0)/2);
    nextP(3,9) = P(3,9) + P(1,9)*SF(7) + P(2,9)*SF(11) + P(4,9)*SF(9) + P(13,9)*SF(15) - P(11,9)*SPP(13) - (P(12,9)*q0)/2 + dt*(P(3,6) + P(1,6)*SF(7) + P(2,6)*SF(11) + P(4,6)*SF(9) + P(13,6)*SF(15) - P(11,6)*SPP(13) - (P(12,6)*q0)/2);
    nextP(3,10) = P(3,10) + P(1,10)*SF(7) + P(2,10)*SF(11) + P(4,10)*SF(9) + P(13,10)*SF(15) - P(11,10)*SPP(13) - (P(12,10)*q0)/2 + dt*(P(3,7) + P(1,7)*SF(7) + P(2,7)*SF(11) + P(4,7)*SF(9) + P(13,7)*SF(15) - P(11,7)*SPP(13) - (P(12,7)*q0)/2);
    nextP(3,11) = P(3,11) + P(1,11)*SF(7) + P(2,11)*SF(11) + P(4,11)*SF(9) + P(13,11)*SF(15) - P(11,11)*SPP(13) - (P(12,11)*q0)/2;
    nextP(3,12) = P(3,12) + P(1,12)*SF(7) + P(2,12)*SF(11) + P(4,12)*SF(9) + P(13,12)*SF(15) - P(11,12)*SPP(13) - (P(12,12)*q0)/2;
    nextP(3,13) = P(3,13) + P(1,13)*SF(7) + P(2,13)*SF(11) + P(4,13)*SF(9) + P(13,13)*SF(15) - P(11,13)*SPP(13) - (P(12,13)*q0)/2;
    nextP(3,14) = P(3,14) + P(1,14)*SF(7) + P(2,14)*SF(11) + P(4,14)*SF(9) + P(13,14)*SF(15) - P(11,14)*SPP(13) - (P(12,14)*q0)/2;
    nextP(3,15) = P(3,15) + P(1,15)*SF(7) + P(2,15)*SF(11) + P(4,15)*SF(9) + P(13,15)*SF(15) - P(11,15)*SPP(13) - (P(12,15)*q0)/2;
    nextP(3,16) = P(3,16) + P(1,16)*SF(7) + P(2,16)*SF(11) + P(4,16)*SF(9) + P(13,16)*SF(15) - P(11,16)*SPP(13) - (P(12,16)*q0)/2;
    nextP(3,17) = P(3,17) + P(1,17)*SF(7) + P(2,17)*SF(11) + P(4,17)*SF(9) + P(13,17)*SF(15) - P(11,17)*SPP(13) - (P(12,17)*q0)/2;
    nextP(3,18) = P(3,18) + P(1,18)*SF(7) + P(2,18)*SF(11) + P(4,18)*SF(9) + P(13,18)*SF(15) - P(11,18)*SPP(13) - (P(12,18)*q0)/2;
    nextP(3,19) = P(3,19) + P(1,19)*SF(7) + P(2,19)*SF(11) + P(4,19)*SF(9) + P(13,19)*SF(15) - P(11,19)*SPP(13) - (P(12,19)*q0)/2;
    nextP(3,20) = P(3,20) + P(1,20)*SF(7) + P(2,20)*SF(11) + P(4,20)*SF(9) + P(13,20)*SF(15) - P(11,20)*SPP(13) - (P(12,20)*q0)/2;
    nextP(3,21) = P(3,21) + P(1,21)*SF(7) + P(2,21)*SF(11) + P(4,21)*SF(9) + P(13,21)*SF(15) - P(11,21)*SPP(13) - (P(12,21)*q0)/2;
    nextP(3,22) = P(3,22) + P(1,22)*SF(7) + P(2,22)*SF(11) + P(4,22)*SF(9) + P(13,22)*SF(15) - P(11,22)*SPP(13) - (P(12,22)*q0)/2;
    nextP(3,23) = P(3,23) + P(1,23)*SF(7) + P(2,23)*SF(11) + P(4,23)*SF(9) + P(13,23)*SF(15) - P(11,23)*SPP(13) - (P(12,23)*q0)/2;
    nextP(3,24) = P(3,24) + P(1,24)*SF(7) + P(2,24)*SF(11) + P(4,24)*SF(9) + P(13,24)*SF(15) - P(11,24)*SPP(13) - (P(12,24)*q0)/2;
    nextP(4,1) = P(4,1) + SQ(7) + P(1,1)*SF(8) + P(2,1)*SF(7) + P(3,1)*SF(10) + P(11,1)*SF(16) - P(12,1)*SF(15) - (P(13,1)*q0)/2 + SF(10)*(P(4,2) + P(1,2)*SF(8) + P(2,2)*SF(7) + P(3,2)*SF(10) + P(11,2)*SF(16) - P(12,2)*SF(15) - (P(13,2)*q0)/2) + SF(12)*(P(4,3) + P(1,3)*SF(8) + P(2,3)*SF(7) + P(3,3)*SF(10) + P(11,3)*SF(16) - P(12,3)*SF(15) - (P(13,3)*q0)/2) + SF(11)*(P(4,4) + P(1,4)*SF(8) + P(2,4)*SF(7) + P(3,4)*SF(10) + P(11,4)*SF(16) - P(12,4)*SF(15) - (P(13,4)*q0)/2) + SF(15)*(P(4,11) + P(1,11)*SF(8) + P(2,11)*SF(7) + P(3,11)*SF(10) + P(11,11)*SF(16) - P(12,11)*SF(15) - (P(13,11)*q0)/2) + SF(16)*(P(4,12) + P(1,12)*SF(8) + P(2,12)*SF(7) + P(3,12)*SF(10) + P(11,12)*SF(16) - P(12,12)*SF(15) - (P(13,12)*q0)/2) + SPP(13)*(P(4,13) + P(1,13)*SF(8) + P(2,13)*SF(7) + P(3,13)*SF(10) + P(11,13)*SF(16) - P(12,13)*SF(15) - (P(13,13)*q0)/2);
    nextP(4,2) = P(4,2) + SQ(5) + P(1,2)*SF(8) + P(2,2)*SF(7) + P(3,2)*SF(10) + P(11,2)*SF(16) - P(12,2)*SF(15) - (P(13,2)*q0)/2 + SF(9)*(P(4,1) + P(1,1)*SF(8) + P(2,1)*SF(7) + P(3,1)*SF(10) + P(11,1)*SF(16) - P(12,1)*SF(15) - (P(13,1)*q0)/2) + SF(8)*(P(4,3) + P(1,3)*SF(8) + P(2,3)*SF(7) + P(3,3)*SF(10) + P(11,3)*SF(16) - P(12,3)*SF(15) - (P(13,3)*q0)/2) + SF(12)*(P(4,4) + P(1,4)*SF(8) + P(2,4)*SF(7) + P(3,4)*SF(10) + P(11,4)*SF(16) - P(12,4)*SF(15) - (P(13,4)*q0)/2) - SF(16)*(P(4,13) + P(1,13)*SF(8) + P(2,13)*SF(7) + P(3,13)*SF(10) + P(11,13)*SF(16) - P(12,13)*SF(15) - (P(13,13)*q0)/2) + SPP(13)*(P(4,12) + P(1,12)*SF(8) + P(2,12)*SF(7) + P(3,12)*SF(10) + P(11,12)*SF(16) - P(12,12)*SF(15) - (P(13,12)*q0)/2) - (q0*(P(4,11) + P(1,11)*SF(8) + P(2,11)*SF(7) + P(3,11)*SF(10) + P(11,11)*SF(16) - P(12,11)*SF(15) - (P(13,11)*q0)/2))/2;
    nextP(4,3) = P(4,3) + SQ(4) + P(1,3)*SF(8) + P(2,3)*SF(7) + P(3,3)*SF(10) + P(11,3)*SF(16) - P(12,3)*SF(15) - (P(13,3)*q0)/2 + SF(7)*(P(4,1) + P(1,1)*SF(8) + P(2,1)*SF(7) + P(3,1)*SF(10) + P(11,1)*SF(16) - P(12,1)*SF(15) - (P(13,1)*q0)/2) + SF(11)*(P(4,2) + P(1,2)*SF(8) + P(2,2)*SF(7) + P(3,2)*SF(10) + P(11,2)*SF(16) - P(12,2)*SF(15) - (P(13,2)*q0)/2) + SF(9)*(P(4,4) + P(1,4)*SF(8) + P(2,4)*SF(7) + P(3,4)*SF(10) + P(11,4)*SF(16) - P(12,4)*SF(15) - (P(13,4)*q0)/2) + SF(15)*(P(4,13) + P(1,13)*SF(8) + P(2,13)*SF(7) + P(3,13)*SF(10) + P(11,13)*SF(16) - P(12,13)*SF(15) - (P(13,13)*q0)/2) - SPP(13)*(P(4,11) + P(1,11)*SF(8) + P(2,11)*SF(7) + P(3,11)*SF(10) + P(11,11)*SF(16) - P(12,11)*SF(15) - (P(13,11)*q0)/2) - (q0*(P(4,12) + P(1,12)*SF(8) + P(2,12)*SF(7) + P(3,12)*SF(10) + P(11,12)*SF(16) - P(12,12)*SF(15) - (P(13,12)*q0)/2))/2;
    nextP(4,4) = P(4,4) + P(1,4)*SF(8) + P(2,4)*SF(7) + P(3,4)*SF(10) + P(11,4)*SF(16) - P(12,4)*SF(15) + (dayCov*SQ(11))/4 + dazCov*SQ(10) - (P(13,4)*q0)/2 + SF(8)*(P(4,1) + P(1,1)*SF(8) + P(2,1)*SF(7) + P(3,1)*SF(10) + P(11,1)*SF(16) - P(12,1)*SF(15) - (P(13,1)*q0)/2) + SF(7)*(P(4,2) + P(1,2)*SF(8) + P(2,2)*SF(7) + P(3,2)*SF(10) + P(11,2)*SF(16) - P(12,2)*SF(15) - (P(13,2)*q0)/2) + SF(10)*(P(4,3) + P(1,3)*SF(8) + P(2,3)*SF(7) + P(3,3)*SF(10) + P(11,3)*SF(16) - P(12,3)*SF(15) - (P(13,3)*q0)/2) + SF(16)*(P(4,11) + P(1,11)*SF(8) + P(2,11)*SF(7) + P(3,11)*SF(10) + P(11,11)*SF(16) - P(12,11)*SF(15) - (P(13,11)*q0)/2) - SF(15)*(P(4,12) + P(1,12)*SF(8) + P(2,12)*SF(7) + P(3,12)*SF(10) + P(11,12)*SF(16) - P(12,12)*SF(15) - (P(13,12)*q0)/2) + (daxCov*q2^2)/4 - (q0*(P(4,13) + P(1,13)*SF(8) + P(2,13)*SF(7) + P(3,13)*SF(10) + P(11,13)*SF(16) - P(12,13)*SF(15) - (P(13,13)*q0)/2))/2;
    nextP(4,5) = P(4,5) + P(1,5)*SF(8) + P(2,5)*SF(7) + P(3,5)*SF(10) + P(11,5)*SF(16) - P(12,5)*SF(15) - (P(13,5)*q0)/2 + SF(6)*(P(4,1) + P(1,1)*SF(8) + P(2,1)*SF(7) + P(3,1)*SF(10) + P(11,1)*SF(16) - P(12,1)*SF(15) - (P(13,1)*q0)/2) + SF(4)*(P(4,2) + P(1,2)*SF(8) + P(2,2)*SF(7) + P(3,2)*SF(10) + P(11,2)*SF(16) - P(12,2)*SF(15) - (P(13,2)*q0)/2) + SPP(1)*(P(4,3) + P(1,3)*SF(8) + P(2,3)*SF(7) + P(3,3)*SF(10) + P(11,3)*SF(16) - P(12,3)*SF(15) - (P(13,3)*q0)/2) - SPP(6)*(P(4,4) + P(1,4)*SF(8) + P(2,4)*SF(7) + P(3,4)*SF(10) + P(11,4)*SF(16) - P(12,4)*SF(15) - (P(13,4)*q0)/2) + SPP(4)*(P(4,14) + P(1,14)*SF(8) + P(2,14)*SF(7) + P(3,14)*SF(10) + P(11,14)*SF(16) - P(12,14)*SF(15) - (P(13,14)*q0)/2) + SPP(9)*(P(4,15) + P(1,15)*SF(8) + P(2,15)*SF(7) + P(3,15)*SF(10) + P(11,15)*SF(16) - P(12,15)*SF(15) - (P(13,15)*q0)/2) - SPP(12)*(P(4,16) + P(1,16)*SF(8) + P(2,16)*SF(7) + P(3,16)*SF(10) + P(11,16)*SF(16) - P(12,16)*SF(15) - (P(13,16)*q0)/2);
    nextP(4,6) = P(4,6) + P(1,6)*SF(8) + P(2,6)*SF(7) + P(3,6)*SF(10) + P(11,6)*SF(16) - P(12,6)*SF(15) - (P(13,6)*q0)/2 + SF(5)*(P(4,1) + P(1,1)*SF(8) + P(2,1)*SF(7) + P(3,1)*SF(10) + P(11,1)*SF(16) - P(12,1)*SF(15) - (P(13,1)*q0)/2) + SF(4)*(P(4,3) + P(1,3)*SF(8) + P(2,3)*SF(7) + P(3,3)*SF(10) + P(11,3)*SF(16) - P(12,3)*SF(15) - (P(13,3)*q0)/2) + SF(6)*(P(4,4) + P(1,4)*SF(8) + P(2,4)*SF(7) + P(3,4)*SF(10) + P(11,4)*SF(16) - P(12,4)*SF(15) - (P(13,4)*q0)/2) - SPP(1)*(P(4,2) + P(1,2)*SF(8) + P(2,2)*SF(7) + P(3,2)*SF(10) + P(11,2)*SF(16) - P(12,2)*SF(15) - (P(13,2)*q0)/2) + SPP(3)*(P(4,15) + P(1,15)*SF(8) + P(2,15)*SF(7) + P(3,15)*SF(10) + P(11,15)*SF(16) - P(12,15)*SF(15) - (P(13,15)*q0)/2) - SPP(11)*(P(4,14) + P(1,14)*SF(8) + P(2,14)*SF(7) + P(3,14)*SF(10) + P(11,14)*SF(16) - P(12,14)*SF(15) - (P(13,14)*q0)/2) + SPP(8)*(P(4,16) + P(1,16)*SF(8) + P(2,16)*SF(7) + P(3,16)*SF(10) + P(11,16)*SF(16) - P(12,16)*SF(15) - (P(13,16)*q0)/2);
    nextP(4,7) = P(4,7) + P(1,7)*SF(8) + P(2,7)*SF(7) + P(3,7)*SF(10) + P(11,7)*SF(16) - P(12,7)*SF(15) - (P(13,7)*q0)/2 + SF(5)*(P(4,2) + P(1,2)*SF(8) + P(2,2)*SF(7) + P(3,2)*SF(10) + P(11,2)*SF(16) - P(12,2)*SF(15) - (P(13,2)*q0)/2) + SF(4)*(P(4,4) + P(1,4)*SF(8) + P(2,4)*SF(7) + P(3,4)*SF(10) + P(11,4)*SF(16) - P(12,4)*SF(15) - (P(13,4)*q0)/2) + SPP(1)*(P(4,1) + P(1,1)*SF(8) + P(2,1)*SF(7) + P(3,1)*SF(10) + P(11,1)*SF(16) - P(12,1)*SF(15) - (P(13,1)*q0)/2) - SPP(5)*(P(4,3) + P(1,3)*SF(8) + P(2,3)*SF(7) + P(3,3)*SF(10) + P(11,3)*SF(16) - P(12,3)*SF(15) - (P(13,3)*q0)/2) + SPP(7)*(P(4,14) + P(1,14)*SF(8) + P(2,14)*SF(7) + P(3,14)*SF(10) + P(11,14)*SF(16) - P(12,14)*SF(15) - (P(13,14)*q0)/2) - SPP(2)*(P(4,16) + P(1,16)*SF(8) + P(2,16)*SF(7) + P(3,16)*SF(10) + P(11,16)*SF(16) - P(12,16)*SF(15) - (P(13,16)*q0)/2) - SPP(10)*(P(4,15) + P(1,15)*SF(8) + P(2,15)*SF(7) + P(3,15)*SF(10) + P(11,15)*SF(16) - P(12,15)*SF(15) - (P(13,15)*q0)/2);
    nextP(4,8) = P(4,8) + P(1,8)*SF(8) + P(2,8)*SF(7) + P(3,8)*SF(10) + P(11,8)*SF(16) - P(12,8)*SF(15) - (P(13,8)*q0)/2 + dt*(P(4,5) + P(1,5)*SF(8) + P(2,5)*SF(7) + P(3,5)*SF(10) + P(11,5)*SF(16) - P(12,5)*SF(15) - (P(13,5)*q0)/2);
    nextP(4,9) = P(4,9) + P(1,9)*SF(8) + P(2,9)*SF(7) + P(3,9)*SF(10) + P(11,9)*SF(16) - P(12,9)*SF(15) - (P(13,9)*q0)/2 + dt*(P(4,6) + P(1,6)*SF(8) + P(2,6)*SF(7) + P(3,6)*SF(10) + P(11,6)*SF(16) - P(12,6)*SF(15) - (P(13,6)*q0)/2);
    nextP(4,10) = P(4,10) + P(1,10)*SF(8) + P(2,10)*SF(7) + P(3,10)*SF(10) + P(11,10)*SF(16) - P(12,10)*SF(15) - (P(13,10)*q0)/2 + dt*(P(4,7) + P(1,7)*SF(8) + P(2,7)*SF(7) + P(3,7)*SF(10) + P(11,7)*SF(16) - P(12,7)*SF(15) - (P(13,7)*q0)/2);
    nextP(4,11) = P(4,11) + P(1,11)*SF(8) + P(2,11)*SF(7) + P(3,11)*SF(10) + P(11,11)*SF(16) - P(12,11)*SF(15) - (P(13,11)*q0)/2;
    nextP(4,12) = P(4,12) + P(1,12)*SF(8) + P(2,12)*SF(7) + P(3,12)*SF(10) + P(11,12)*SF(16) - P(12,12)*SF(15) - (P(13,12)*q0)/2;
    nextP(4,13) = P(4,13) + P(1,13)*SF(8) + P(2,13)*SF(7) + P(3,13)*SF(10) + P(11,13)*SF(16) - P(12,13)*SF(15) - (P(13,13)*q0)/2;
    nextP(4,14) = P(4,14) + P(1,14)*SF(8) + P(2,14)*SF(7) + P(3,14)*SF(10) + P(11,14)*SF(16) - P(12,14)*SF(15) - (P(13,14)*q0)/2;
    nextP(4,15) = P(4,15) + P(1,15)*SF(8) + P(2,15)*SF(7) + P(3,15)*SF(10) + P(11,15)*SF(16) - P(12,15)*SF(15) - (P(13,15)*q0)/2;
    nextP(4,16) = P(4,16) + P(1,16)*SF(8) + P(2,16)*SF(7) + P(3,16)*SF(10) + P(11,16)*SF(16) - P(12,16)*SF(15) - (P(13,16)*q0)/2;
    nextP(4,17) = P(4,17) + P(1,17)*SF(8) + P(2,17)*SF(7) + P(3,17)*SF(10) + P(11,17)*SF(16) - P(12,17)*SF(15) - (P(13,17)*q0)/2;
    nextP(4,18) = P(4,18) + P(1,18)*SF(8) + P(2,18)*SF(7) + P(3,18)*SF(10) + P(11,18)*SF(16) - P(12,18)*SF(15) - (P(13,18)*q0)/2;
    nextP(4,19) = P(4,19) + P(1,19)*SF(8) + P(2,19)*SF(7) + P(3,19)*SF(10) + P(11,19)*SF(16) - P(12,19)*SF(15) - (P(13,19)*q0)/2;
    nextP(4,20) = P(4,20) + P(1,20)*SF(8) + P(2,20)*SF(7) + P(3,20)*SF(10) + P(11,20)*SF(16) - P(12,20)*SF(15) - (P(13,20)*q0)/2;
    nextP(4,21) = P(4,21) + P(1,21)*SF(8) + P(2,21)*SF(7) + P(3,21)*SF(10) + P(11,21)*SF(16) - P(12,21)*SF(15) - (P(13,21)*q0)/2;
    nextP(4,22) = P(4,22) + P(1,22)*SF(8) + P(2,22)*SF(7) + P(3,22)*SF(10) + P(11,22)*SF(16) - P(12,22)*SF(15) - (P(13,22)*q0)/2;
    nextP(4,23) = P(4,23) + P(1,23)*SF(8) + P(2,23)*SF(7) + P(3,23)*SF(10) + P(11,23)*SF(16) - P(12,23)*SF(15) - (P(13,23)*q0)/2;
    nextP(4,24) = P(4,24) + P(1,24)*SF(8) + P(2,24)*SF(7) + P(3,24)*SF(10) + P(11,24)*SF(16) - P(12,24)*SF(15) - (P(13,24)*q0)/2;
    nextP(5,1) = P(5,1) + P(1,1)*SF(6) + P(2,1)*SF(4) + P(3,1)*SPP(1) - P(4,1)*SPP(6) + P(14,1)*SPP(4) + P(15,1)*SPP(9) - P(16,1)*SPP(12) + SF(10)*(P(5,2) + P(1,2)*SF(6) + P(2,2)*SF(4) + P(3,2)*SPP(1) - P(4,2)*SPP(6) + P(14,2)*SPP(4) + P(15,2)*SPP(9) - P(16,2)*SPP(12)) + SF(12)*(P(5,3) + P(1,3)*SF(6) + P(2,3)*SF(4) + P(3,3)*SPP(1) - P(4,3)*SPP(6) + P(14,3)*SPP(4) + P(15,3)*SPP(9) - P(16,3)*SPP(12)) + SF(11)*(P(5,4) + P(1,4)*SF(6) + P(2,4)*SF(4) + P(3,4)*SPP(1) - P(4,4)*SPP(6) + P(14,4)*SPP(4) + P(15,4)*SPP(9) - P(16,4)*SPP(12)) + SF(15)*(P(5,11) + P(1,11)*SF(6) + P(2,11)*SF(4) + P(3,11)*SPP(1) - P(4,11)*SPP(6) + P(14,11)*SPP(4) + P(15,11)*SPP(9) - P(16,11)*SPP(12)) + SF(16)*(P(5,12) + P(1,12)*SF(6) + P(2,12)*SF(4) + P(3,12)*SPP(1) - P(4,12)*SPP(6) + P(14,12)*SPP(4) + P(15,12)*SPP(9) - P(16,12)*SPP(12)) + SPP(13)*(P(5,13) + P(1,13)*SF(6) + P(2,13)*SF(4) + P(3,13)*SPP(1) - P(4,13)*SPP(6) + P(14,13)*SPP(4) + P(15,13)*SPP(9) - P(16,13)*SPP(12));
    nextP(5,2) = P(5,2) + P(1,2)*SF(6) + P(2,2)*SF(4) + P(3,2)*SPP(1) - P(4,2)*SPP(6) + P(14,2)*SPP(4) + P(15,2)*SPP(9) - P(16,2)*SPP(12) + SF(9)*(P(5,1) + P(1,1)*SF(6) + P(2,1)*SF(4) + P(3,1)*SPP(1) - P(4,1)*SPP(6) + P(14,1)*SPP(4) + P(15,1)*SPP(9) - P(16,1)*SPP(12)) + SF(8)*(P(5,3) + P(1,3)*SF(6) + P(2,3)*SF(4) + P(3,3)*SPP(1) - P(4,3)*SPP(6) + P(14,3)*SPP(4) + P(15,3)*SPP(9) - P(16,3)*SPP(12)) + SF(12)*(P(5,4) + P(1,4)*SF(6) + P(2,4)*SF(4) + P(3,4)*SPP(1) - P(4,4)*SPP(6) + P(14,4)*SPP(4) + P(15,4)*SPP(9) - P(16,4)*SPP(12)) - SF(16)*(P(5,13) + P(1,13)*SF(6) + P(2,13)*SF(4) + P(3,13)*SPP(1) - P(4,13)*SPP(6) + P(14,13)*SPP(4) + P(15,13)*SPP(9) - P(16,13)*SPP(12)) + SPP(13)*(P(5,12) + P(1,12)*SF(6) + P(2,12)*SF(4) + P(3,12)*SPP(1) - P(4,12)*SPP(6) + P(14,12)*SPP(4) + P(15,12)*SPP(9) - P(16,12)*SPP(12)) - (q0*(P(5,11) + P(1,11)*SF(6) + P(2,11)*SF(4) + P(3,11)*SPP(1) - P(4,11)*SPP(6) + P(14,11)*SPP(4) + P(15,11)*SPP(9) - P(16,11)*SPP(12)))/2;
    nextP(5,3) = P(5,3) + P(1,3)*SF(6) + P(2,3)*SF(4) + P(3,3)*SPP(1) - P(4,3)*SPP(6) + P(14,3)*SPP(4) + P(15,3)*SPP(9) - P(16,3)*SPP(12) + SF(7)*(P(5,1) + P(1,1)*SF(6) + P(2,1)*SF(4) + P(3,1)*SPP(1) - P(4,1)*SPP(6) + P(14,1)*SPP(4) + P(15,1)*SPP(9) - P(16,1)*SPP(12)) + SF(11)*(P(5,2) + P(1,2)*SF(6) + P(2,2)*SF(4) + P(3,2)*SPP(1) - P(4,2)*SPP(6) + P(14,2)*SPP(4) + P(15,2)*SPP(9) - P(16,2)*SPP(12)) + SF(9)*(P(5,4) + P(1,4)*SF(6) + P(2,4)*SF(4) + P(3,4)*SPP(1) - P(4,4)*SPP(6) + P(14,4)*SPP(4) + P(15,4)*SPP(9) - P(16,4)*SPP(12)) + SF(15)*(P(5,13) + P(1,13)*SF(6) + P(2,13)*SF(4) + P(3,13)*SPP(1) - P(4,13)*SPP(6) + P(14,13)*SPP(4) + P(15,13)*SPP(9) - P(16,13)*SPP(12)) - SPP(13)*(P(5,11) + P(1,11)*SF(6) + P(2,11)*SF(4) + P(3,11)*SPP(1) - P(4,11)*SPP(6) + P(14,11)*SPP(4) + P(15,11)*SPP(9) - P(16,11)*SPP(12)) - (q0*(P(5,12) + P(1,12)*SF(6) + P(2,12)*SF(4) + P(3,12)*SPP(1) - P(4,12)*SPP(6) + P(14,12)*SPP(4) + P(15,12)*SPP(9) - P(16,12)*SPP(12)))/2;
    nextP(5,4) = P(5,4) + P(1,4)*SF(6) + P(2,4)*SF(4) + P(3,4)*SPP(1) - P(4,4)*SPP(6) + P(14,4)*SPP(4) + P(15,4)*SPP(9) - P(16,4)*SPP(12) + SF(8)*(P(5,1) + P(1,1)*SF(6) + P(2,1)*SF(4) + P(3,1)*SPP(1) - P(4,1)*SPP(6) + P(14,1)*SPP(4) + P(15,1)*SPP(9) - P(16,1)*SPP(12)) + SF(7)*(P(5,2) + P(1,2)*SF(6) + P(2,2)*SF(4) + P(3,2)*SPP(1) - P(4,2)*SPP(6) + P(14,2)*SPP(4) + P(15,2)*SPP(9) - P(16,2)*SPP(12)) + SF(10)*(P(5,3) + P(1,3)*SF(6) + P(2,3)*SF(4) + P(3,3)*SPP(1) - P(4,3)*SPP(6) + P(14,3)*SPP(4) + P(15,3)*SPP(9) - P(16,3)*SPP(12)) + SF(16)*(P(5,11) + P(1,11)*SF(6) + P(2,11)*SF(4) + P(3,11)*SPP(1) - P(4,11)*SPP(6) + P(14,11)*SPP(4) + P(15,11)*SPP(9) - P(16,11)*SPP(12)) - SF(15)*(P(5,12) + P(1,12)*SF(6) + P(2,12)*SF(4) + P(3,12)*SPP(1) - P(4,12)*SPP(6) + P(14,12)*SPP(4) + P(15,12)*SPP(9) - P(16,12)*SPP(12)) - (q0*(P(5,13) + P(1,13)*SF(6) + P(2,13)*SF(4) + P(3,13)*SPP(1) - P(4,13)*SPP(6) + P(14,13)*SPP(4) + P(15,13)*SPP(9) - P(16,13)*SPP(12)))/2;
    nextP(5,5) = P(5,5) + P(1,5)*SF(6) + P(2,5)*SF(4) + P(3,5)*SPP(1) - P(4,5)*SPP(6) + P(14,5)*SPP(4) + P(15,5)*SPP(9) - P(16,5)*SPP(12) + dvyCov*(SG(8) - 2*q0*q3)^2 + dvzCov*(SG(7) + 2*q0*q2)^2 + SF(6)*(P(5,1) + P(1,1)*SF(6) + P(2,1)*SF(4) + P(3,1)*SPP(1) - P(4,1)*SPP(6) + P(14,1)*SPP(4) + P(15,1)*SPP(9) - P(16,1)*SPP(12)) + SF(4)*(P(5,2) + P(1,2)*SF(6) + P(2,2)*SF(4) + P(3,2)*SPP(1) - P(4,2)*SPP(6) + P(14,2)*SPP(4) + P(15,2)*SPP(9) - P(16,2)*SPP(12)) + SPP(1)*(P(5,3) + P(1,3)*SF(6) + P(2,3)*SF(4) + P(3,3)*SPP(1) - P(4,3)*SPP(6) + P(14,3)*SPP(4) + P(15,3)*SPP(9) - P(16,3)*SPP(12)) - SPP(6)*(P(5,4) + P(1,4)*SF(6) + P(2,4)*SF(4) + P(3,4)*SPP(1) - P(4,4)*SPP(6) + P(14,4)*SPP(4) + P(15,4)*SPP(9) - P(16,4)*SPP(12)) + SPP(4)*(P(5,14) + P(1,14)*SF(6) + P(2,14)*SF(4) + P(3,14)*SPP(1) - P(4,14)*SPP(6) + P(14,14)*SPP(4) + P(15,14)*SPP(9) - P(16,14)*SPP(12)) + SPP(9)*(P(5,15) + P(1,15)*SF(6) + P(2,15)*SF(4) + P(3,15)*SPP(1) - P(4,15)*SPP(6) + P(14,15)*SPP(4) + P(15,15)*SPP(9) - P(16,15)*SPP(12)) - SPP(12)*(P(5,16) + P(1,16)*SF(6) + P(2,16)*SF(4) + P(3,16)*SPP(1) - P(4,16)*SPP(6) + P(14,16)*SPP(4) + P(15,16)*SPP(9) - P(16,16)*SPP(12)) + dvxCov*(SG(2) + SG(3) - SG(4) - SG(5))^2;
    nextP(5,6) = P(5,6) + SQ(3) + P(1,6)*SF(6) + P(2,6)*SF(4) + P(3,6)*SPP(1) - P(4,6)*SPP(6) + P(14,6)*SPP(4) + P(15,6)*SPP(9) - P(16,6)*SPP(12) + SF(5)*(P(5,1) + P(1,1)*SF(6) + P(2,1)*SF(4) + P(3,1)*SPP(1) - P(4,1)*SPP(6) + P(14,1)*SPP(4) + P(15,1)*SPP(9) - P(16,1)*SPP(12)) + SF(4)*(P(5,3) + P(1,3)*SF(6) + P(2,3)*SF(4) + P(3,3)*SPP(1) - P(4,3)*SPP(6) + P(14,3)*SPP(4) + P(15,3)*SPP(9) - P(16,3)*SPP(12)) + SF(6)*(P(5,4) + P(1,4)*SF(6) + P(2,4)*SF(4) + P(3,4)*SPP(1) - P(4,4)*SPP(6) + P(14,4)*SPP(4) + P(15,4)*SPP(9) - P(16,4)*SPP(12)) - SPP(1)*(P(5,2) + P(1,2)*SF(6) + P(2,2)*SF(4) + P(3,2)*SPP(1) - P(4,2)*SPP(6) + P(14,2)*SPP(4) + P(15,2)*SPP(9) - P(16,2)*SPP(12)) + SPP(3)*(P(5,15) + P(1,15)*SF(6) + P(2,15)*SF(4) + P(3,15)*SPP(1) - P(4,15)*SPP(6) + P(14,15)*SPP(4) + P(15,15)*SPP(9) - P(16,15)*SPP(12)) - SPP(11)*(P(5,14) + P(1,14)*SF(6) + P(2,14)*SF(4) + P(3,14)*SPP(1) - P(4,14)*SPP(6) + P(14,14)*SPP(4) + P(15,14)*SPP(9) - P(16,14)*SPP(12)) + SPP(8)*(P(5,16) + P(1,16)*SF(6) + P(2,16)*SF(4) + P(3,16)*SPP(1) - P(4,16)*SPP(6) + P(14,16)*SPP(4) + P(15,16)*SPP(9) - P(16,16)*SPP(12));
    nextP(5,7) = P(5,7) + SQ(2) + P(1,7)*SF(6) + P(2,7)*SF(4) + P(3,7)*SPP(1) - P(4,7)*SPP(6) + P(14,7)*SPP(4) + P(15,7)*SPP(9) - P(16,7)*SPP(12) + SF(5)*(P(5,2) + P(1,2)*SF(6) + P(2,2)*SF(4) + P(3,2)*SPP(1) - P(4,2)*SPP(6) + P(14,2)*SPP(4) + P(15,2)*SPP(9) - P(16,2)*SPP(12)) + SF(4)*(P(5,4) + P(1,4)*SF(6) + P(2,4)*SF(4) + P(3,4)*SPP(1) - P(4,4)*SPP(6) + P(14,4)*SPP(4) + P(15,4)*SPP(9) - P(16,4)*SPP(12)) + SPP(1)*(P(5,1) + P(1,1)*SF(6) + P(2,1)*SF(4) + P(3,1)*SPP(1) - P(4,1)*SPP(6) + P(14,1)*SPP(4) + P(15,1)*SPP(9) - P(16,1)*SPP(12)) - SPP(5)*(P(5,3) + P(1,3)*SF(6) + P(2,3)*SF(4) + P(3,3)*SPP(1) - P(4,3)*SPP(6) + P(14,3)*SPP(4) + P(15,3)*SPP(9) - P(16,3)*SPP(12)) + SPP(7)*(P(5,14) + P(1,14)*SF(6) + P(2,14)*SF(4) + P(3,14)*SPP(1) - P(4,14)*SPP(6) + P(14,14)*SPP(4) + P(15,14)*SPP(9) - P(16,14)*SPP(12)) - SPP(2)*(P(5,16) + P(1,16)*SF(6) + P(2,16)*SF(4) + P(3,16)*SPP(1) - P(4,16)*SPP(6) + P(14,16)*SPP(4) + P(15,16)*SPP(9) - P(16,16)*SPP(12)) - SPP(10)*(P(5,15) + P(1,15)*SF(6) + P(2,15)*SF(4) + P(3,15)*SPP(1) - P(4,15)*SPP(6) + P(14,15)*SPP(4) + P(15,15)*SPP(9) - P(16,15)*SPP(12));
    nextP(5,8) = P(5,8) + P(1,8)*SF(6) + P(2,8)*SF(4) + P(3,8)*SPP(1) - P(4,8)*SPP(6) + P(14,8)*SPP(4) + P(15,8)*SPP(9) - P(16,8)*SPP(12) + dt*(P(5,5) + P(1,5)*SF(6) + P(2,5)*SF(4) + P(3,5)*SPP(1) - P(4,5)*SPP(6) + P(14,5)*SPP(4) + P(15,5)*SPP(9) - P(16,5)*SPP(12));
    nextP(5,9) = P(5,9) + P(1,9)*SF(6) + P(2,9)*SF(4) + P(3,9)*SPP(1) - P(4,9)*SPP(6) + P(14,9)*SPP(4) + P(15,9)*SPP(9) - P(16,9)*SPP(12) + dt*(P(5,6) + P(1,6)*SF(6) + P(2,6)*SF(4) + P(3,6)*SPP(1) - P(4,6)*SPP(6) + P(14,6)*SPP(4) + P(15,6)*SPP(9) - P(16,6)*SPP(12));
    nextP(5,10) = P(5,10) + P(1,10)*SF(6) + P(2,10)*SF(4) + P(3,10)*SPP(1) - P(4,10)*SPP(6) + P(14,10)*SPP(4) + P(15,10)*SPP(9) - P(16,10)*SPP(12) + dt*(P(5,7) + P(1,7)*SF(6) + P(2,7)*SF(4) + P(3,7)*SPP(1) - P(4,7)*SPP(6) + P(14,7)*SPP(4) + P(15,7)*SPP(9) - P(16,7)*SPP(12));
    nextP(5,11) = P(5,11) + P(1,11)*SF(6) + P(2,11)*SF(4) + P(3,11)*SPP(1) - P(4,11)*SPP(6) + P(14,11)*SPP(4) + P(15,11)*SPP(9) - P(16,11)*SPP(12);
    nextP(5,12) = P(5,12) + P(1,12)*SF(6) + P(2,12)*SF(4) + P(3,12)*SPP(1) - P(4,12)*SPP(6) + P(14,12)*SPP(4) + P(15,12)*SPP(9) - P(16,12)*SPP(12);
    nextP(5,13) = P(5,13) + P(1,13)*SF(6) + P(2,13)*SF(4) + P(3,13)*SPP(1) - P(4,13)*SPP(6) + P(14,13)*SPP(4) + P(15,13)*SPP(9) - P(16,13)*SPP(12);
    nextP(5,14) = P(5,14) + P(1,14)*SF(6) + P(2,14)*SF(4) + P(3,14)*SPP(1) - P(4,14)*SPP(6) + P(14,14)*SPP(4) + P(15,14)*SPP(9) - P(16,14)*SPP(12);
    nextP(5,15) = P(5,15) + P(1,15)*SF(6) + P(2,15)*SF(4) + P(3,15)*SPP(1) - P(4,15)*SPP(6) + P(14,15)*SPP(4) + P(15,15)*SPP(9) - P(16,15)*SPP(12);
    nextP(5,16) = P(5,16) + P(1,16)*SF(6) + P(2,16)*SF(4) + P(3,16)*SPP(1) - P(4,16)*SPP(6) + P(14,16)*SPP(4) + P(15,16)*SPP(9) - P(16,16)*SPP(12);
    nextP(5,17) = P(5,17) + P(1,17)*SF(6) + P(2,17)*SF(4) + P(3,17)*SPP(1) - P(4,17)*SPP(6) + P(14,17)*SPP(4) + P(15,17)*SPP(9) - P(16,17)*SPP(12);
    nextP(5,18) = P(5,18) + P(1,18)*SF(6) + P(2,18)*SF(4) + P(3,18)*SPP(1) - P(4,18)*SPP(6) + P(14,18)*SPP(4) + P(15,18)*SPP(9) - P(16,18)*SPP(12);
    nextP(5,19) = P(5,19) + P(1,19)*SF(6) + P(2,19)*SF(4) + P(3,19)*SPP(1) - P(4,19)*SPP(6) + P(14,19)*SPP(4) + P(15,19)*SPP(9) - P(16,19)*SPP(12);
    nextP(5,20) = P(5,20) + P(1,20)*SF(6) + P(2,20)*SF(4) + P(3,20)*SPP(1) - P(4,20)*SPP(6) + P(14,20)*SPP(4) + P(15,20)*SPP(9) - P(16,20)*SPP(12);
    nextP(5,21) = P(5,21) + P(1,21)*SF(6) + P(2,21)*SF(4) + P(3,21)*SPP(1) - P(4,21)*SPP(6) + P(14,21)*SPP(4) + P(15,21)*SPP(9) - P(16,21)*SPP(12);
    nextP(5,22) = P(5,22) + P(1,22)*SF(6) + P(2,22)*SF(4) + P(3,22)*SPP(1) - P(4,22)*SPP(6) + P(14,22)*SPP(4) + P(15,22)*SPP(9) - P(16,22)*SPP(12);
    nextP(5,23) = P(5,23) + P(1,23)*SF(6) + P(2,23)*SF(4) + P(3,23)*SPP(1) - P(4,23)*SPP(6) + P(14,23)*SPP(4) + P(15,23)*SPP(9) - P(16,23)*SPP(12);
    nextP(5,24) = P(5,24) + P(1,24)*SF(6) + P(2,24)*SF(4) + P(3,24)*SPP(1) - P(4,24)*SPP(6) + P(14,24)*SPP(4) + P(15,24)*SPP(9) - P(16,24)*SPP(12);
    nextP(6,1) = P(6,1) + P(1,1)*SF(5) + P(3,1)*SF(4) + P(4,1)*SF(6) - P(2,1)*SPP(1) - P(14,1)*SPP(11) + P(15,1)*SPP(3) + P(16,1)*SPP(8) + SF(10)*(P(6,2) + P(1,2)*SF(5) + P(3,2)*SF(4) + P(4,2)*SF(6) - P(2,2)*SPP(1) - P(14,2)*SPP(11) + P(15,2)*SPP(3) + P(16,2)*SPP(8)) + SF(12)*(P(6,3) + P(1,3)*SF(5) + P(3,3)*SF(4) + P(4,3)*SF(6) - P(2,3)*SPP(1) - P(14,3)*SPP(11) + P(15,3)*SPP(3) + P(16,3)*SPP(8)) + SF(11)*(P(6,4) + P(1,4)*SF(5) + P(3,4)*SF(4) + P(4,4)*SF(6) - P(2,4)*SPP(1) - P(14,4)*SPP(11) + P(15,4)*SPP(3) + P(16,4)*SPP(8)) + SF(15)*(P(6,11) + P(1,11)*SF(5) + P(3,11)*SF(4) + P(4,11)*SF(6) - P(2,11)*SPP(1) - P(14,11)*SPP(11) + P(15,11)*SPP(3) + P(16,11)*SPP(8)) + SF(16)*(P(6,12) + P(1,12)*SF(5) + P(3,12)*SF(4) + P(4,12)*SF(6) - P(2,12)*SPP(1) - P(14,12)*SPP(11) + P(15,12)*SPP(3) + P(16,12)*SPP(8)) + SPP(13)*(P(6,13) + P(1,13)*SF(5) + P(3,13)*SF(4) + P(4,13)*SF(6) - P(2,13)*SPP(1) - P(14,13)*SPP(11) + P(15,13)*SPP(3) + P(16,13)*SPP(8));
    nextP(6,2) = P(6,2) + P(1,2)*SF(5) + P(3,2)*SF(4) + P(4,2)*SF(6) - P(2,2)*SPP(1) - P(14,2)*SPP(11) + P(15,2)*SPP(3) + P(16,2)*SPP(8) + SF(9)*(P(6,1) + P(1,1)*SF(5) + P(3,1)*SF(4) + P(4,1)*SF(6) - P(2,1)*SPP(1) - P(14,1)*SPP(11) + P(15,1)*SPP(3) + P(16,1)*SPP(8)) + SF(8)*(P(6,3) + P(1,3)*SF(5) + P(3,3)*SF(4) + P(4,3)*SF(6) - P(2,3)*SPP(1) - P(14,3)*SPP(11) + P(15,3)*SPP(3) + P(16,3)*SPP(8)) + SF(12)*(P(6,4) + P(1,4)*SF(5) + P(3,4)*SF(4) + P(4,4)*SF(6) - P(2,4)*SPP(1) - P(14,4)*SPP(11) + P(15,4)*SPP(3) + P(16,4)*SPP(8)) - SF(16)*(P(6,13) + P(1,13)*SF(5) + P(3,13)*SF(4) + P(4,13)*SF(6) - P(2,13)*SPP(1) - P(14,13)*SPP(11) + P(15,13)*SPP(3) + P(16,13)*SPP(8)) + SPP(13)*(P(6,12) + P(1,12)*SF(5) + P(3,12)*SF(4) + P(4,12)*SF(6) - P(2,12)*SPP(1) - P(14,12)*SPP(11) + P(15,12)*SPP(3) + P(16,12)*SPP(8)) - (q0*(P(6,11) + P(1,11)*SF(5) + P(3,11)*SF(4) + P(4,11)*SF(6) - P(2,11)*SPP(1) - P(14,11)*SPP(11) + P(15,11)*SPP(3) + P(16,11)*SPP(8)))/2;
    nextP(6,3) = P(6,3) + P(1,3)*SF(5) + P(3,3)*SF(4) + P(4,3)*SF(6) - P(2,3)*SPP(1) - P(14,3)*SPP(11) + P(15,3)*SPP(3) + P(16,3)*SPP(8) + SF(7)*(P(6,1) + P(1,1)*SF(5) + P(3,1)*SF(4) + P(4,1)*SF(6) - P(2,1)*SPP(1) - P(14,1)*SPP(11) + P(15,1)*SPP(3) + P(16,1)*SPP(8)) + SF(11)*(P(6,2) + P(1,2)*SF(5) + P(3,2)*SF(4) + P(4,2)*SF(6) - P(2,2)*SPP(1) - P(14,2)*SPP(11) + P(15,2)*SPP(3) + P(16,2)*SPP(8)) + SF(9)*(P(6,4) + P(1,4)*SF(5) + P(3,4)*SF(4) + P(4,4)*SF(6) - P(2,4)*SPP(1) - P(14,4)*SPP(11) + P(15,4)*SPP(3) + P(16,4)*SPP(8)) + SF(15)*(P(6,13) + P(1,13)*SF(5) + P(3,13)*SF(4) + P(4,13)*SF(6) - P(2,13)*SPP(1) - P(14,13)*SPP(11) + P(15,13)*SPP(3) + P(16,13)*SPP(8)) - SPP(13)*(P(6,11) + P(1,11)*SF(5) + P(3,11)*SF(4) + P(4,11)*SF(6) - P(2,11)*SPP(1) - P(14,11)*SPP(11) + P(15,11)*SPP(3) + P(16,11)*SPP(8)) - (q0*(P(6,12) + P(1,12)*SF(5) + P(3,12)*SF(4) + P(4,12)*SF(6) - P(2,12)*SPP(1) - P(14,12)*SPP(11) + P(15,12)*SPP(3) + P(16,12)*SPP(8)))/2;
    nextP(6,4) = P(6,4) + P(1,4)*SF(5) + P(3,4)*SF(4) + P(4,4)*SF(6) - P(2,4)*SPP(1) - P(14,4)*SPP(11) + P(15,4)*SPP(3) + P(16,4)*SPP(8) + SF(8)*(P(6,1) + P(1,1)*SF(5) + P(3,1)*SF(4) + P(4,1)*SF(6) - P(2,1)*SPP(1) - P(14,1)*SPP(11) + P(15,1)*SPP(3) + P(16,1)*SPP(8)) + SF(7)*(P(6,2) + P(1,2)*SF(5) + P(3,2)*SF(4) + P(4,2)*SF(6) - P(2,2)*SPP(1) - P(14,2)*SPP(11) + P(15,2)*SPP(3) + P(16,2)*SPP(8)) + SF(10)*(P(6,3) + P(1,3)*SF(5) + P(3,3)*SF(4) + P(4,3)*SF(6) - P(2,3)*SPP(1) - P(14,3)*SPP(11) + P(15,3)*SPP(3) + P(16,3)*SPP(8)) + SF(16)*(P(6,11) + P(1,11)*SF(5) + P(3,11)*SF(4) + P(4,11)*SF(6) - P(2,11)*SPP(1) - P(14,11)*SPP(11) + P(15,11)*SPP(3) + P(16,11)*SPP(8)) - SF(15)*(P(6,12) + P(1,12)*SF(5) + P(3,12)*SF(4) + P(4,12)*SF(6) - P(2,12)*SPP(1) - P(14,12)*SPP(11) + P(15,12)*SPP(3) + P(16,12)*SPP(8)) - (q0*(P(6,13) + P(1,13)*SF(5) + P(3,13)*SF(4) + P(4,13)*SF(6) - P(2,13)*SPP(1) - P(14,13)*SPP(11) + P(15,13)*SPP(3) + P(16,13)*SPP(8)))/2;
    nextP(6,5) = P(6,5) + SQ(3) + P(1,5)*SF(5) + P(3,5)*SF(4) + P(4,5)*SF(6) - P(2,5)*SPP(1) - P(14,5)*SPP(11) + P(15,5)*SPP(3) + P(16,5)*SPP(8) + SF(6)*(P(6,1) + P(1,1)*SF(5) + P(3,1)*SF(4) + P(4,1)*SF(6) - P(2,1)*SPP(1) - P(14,1)*SPP(11) + P(15,1)*SPP(3) + P(16,1)*SPP(8)) + SF(4)*(P(6,2) + P(1,2)*SF(5) + P(3,2)*SF(4) + P(4,2)*SF(6) - P(2,2)*SPP(1) - P(14,2)*SPP(11) + P(15,2)*SPP(3) + P(16,2)*SPP(8)) + SPP(1)*(P(6,3) + P(1,3)*SF(5) + P(3,3)*SF(4) + P(4,3)*SF(6) - P(2,3)*SPP(1) - P(14,3)*SPP(11) + P(15,3)*SPP(3) + P(16,3)*SPP(8)) - SPP(6)*(P(6,4) + P(1,4)*SF(5) + P(3,4)*SF(4) + P(4,4)*SF(6) - P(2,4)*SPP(1) - P(14,4)*SPP(11) + P(15,4)*SPP(3) + P(16,4)*SPP(8)) + SPP(4)*(P(6,14) + P(1,14)*SF(5) + P(3,14)*SF(4) + P(4,14)*SF(6) - P(2,14)*SPP(1) - P(14,14)*SPP(11) + P(15,14)*SPP(3) + P(16,14)*SPP(8)) + SPP(9)*(P(6,15) + P(1,15)*SF(5) + P(3,15)*SF(4) + P(4,15)*SF(6) - P(2,15)*SPP(1) - P(14,15)*SPP(11) + P(15,15)*SPP(3) + P(16,15)*SPP(8)) - SPP(12)*(P(6,16) + P(1,16)*SF(5) + P(3,16)*SF(4) + P(4,16)*SF(6) - P(2,16)*SPP(1) - P(14,16)*SPP(11) + P(15,16)*SPP(3) + P(16,16)*SPP(8));
    nextP(6,6) = P(6,6) + P(1,6)*SF(5) + P(3,6)*SF(4) + P(4,6)*SF(6) - P(2,6)*SPP(1) - P(14,6)*SPP(11) + P(15,6)*SPP(3) + P(16,6)*SPP(8) + dvxCov*(SG(8) + 2*q0*q3)^2 + dvzCov*(SG(6) - 2*q0*q1)^2 + SF(5)*(P(6,1) + P(1,1)*SF(5) + P(3,1)*SF(4) + P(4,1)*SF(6) - P(2,1)*SPP(1) - P(14,1)*SPP(11) + P(15,1)*SPP(3) + P(16,1)*SPP(8)) + SF(4)*(P(6,3) + P(1,3)*SF(5) + P(3,3)*SF(4) + P(4,3)*SF(6) - P(2,3)*SPP(1) - P(14,3)*SPP(11) + P(15,3)*SPP(3) + P(16,3)*SPP(8)) + SF(6)*(P(6,4) + P(1,4)*SF(5) + P(3,4)*SF(4) + P(4,4)*SF(6) - P(2,4)*SPP(1) - P(14,4)*SPP(11) + P(15,4)*SPP(3) + P(16,4)*SPP(8)) - SPP(1)*(P(6,2) + P(1,2)*SF(5) + P(3,2)*SF(4) + P(4,2)*SF(6) - P(2,2)*SPP(1) - P(14,2)*SPP(11) + P(15,2)*SPP(3) + P(16,2)*SPP(8)) + SPP(3)*(P(6,15) + P(1,15)*SF(5) + P(3,15)*SF(4) + P(4,15)*SF(6) - P(2,15)*SPP(1) - P(14,15)*SPP(11) + P(15,15)*SPP(3) + P(16,15)*SPP(8)) - SPP(11)*(P(6,14) + P(1,14)*SF(5) + P(3,14)*SF(4) + P(4,14)*SF(6) - P(2,14)*SPP(1) - P(14,14)*SPP(11) + P(15,14)*SPP(3) + P(16,14)*SPP(8)) + SPP(8)*(P(6,16) + P(1,16)*SF(5) + P(3,16)*SF(4) + P(4,16)*SF(6) - P(2,16)*SPP(1) - P(14,16)*SPP(11) + P(15,16)*SPP(3) + P(16,16)*SPP(8)) + dvyCov*(SG(2) - SG(3) + SG(4) - SG(5))^2;
    nextP(6,7) = P(6,7) + SQ(1) + P(1,7)*SF(5) + P(3,7)*SF(4) + P(4,7)*SF(6) - P(2,7)*SPP(1) - P(14,7)*SPP(11) + P(15,7)*SPP(3) + P(16,7)*SPP(8) + SF(5)*(P(6,2) + P(1,2)*SF(5) + P(3,2)*SF(4) + P(4,2)*SF(6) - P(2,2)*SPP(1) - P(14,2)*SPP(11) + P(15,2)*SPP(3) + P(16,2)*SPP(8)) + SF(4)*(P(6,4) + P(1,4)*SF(5) + P(3,4)*SF(4) + P(4,4)*SF(6) - P(2,4)*SPP(1) - P(14,4)*SPP(11) + P(15,4)*SPP(3) + P(16,4)*SPP(8)) + SPP(1)*(P(6,1) + P(1,1)*SF(5) + P(3,1)*SF(4) + P(4,1)*SF(6) - P(2,1)*SPP(1) - P(14,1)*SPP(11) + P(15,1)*SPP(3) + P(16,1)*SPP(8)) - SPP(5)*(P(6,3) + P(1,3)*SF(5) + P(3,3)*SF(4) + P(4,3)*SF(6) - P(2,3)*SPP(1) - P(14,3)*SPP(11) + P(15,3)*SPP(3) + P(16,3)*SPP(8)) + SPP(7)*(P(6,14) + P(1,14)*SF(5) + P(3,14)*SF(4) + P(4,14)*SF(6) - P(2,14)*SPP(1) - P(14,14)*SPP(11) + P(15,14)*SPP(3) + P(16,14)*SPP(8)) - SPP(2)*(P(6,16) + P(1,16)*SF(5) + P(3,16)*SF(4) + P(4,16)*SF(6) - P(2,16)*SPP(1) - P(14,16)*SPP(11) + P(15,16)*SPP(3) + P(16,16)*SPP(8)) - SPP(10)*(P(6,15) + P(1,15)*SF(5) + P(3,15)*SF(4) + P(4,15)*SF(6) - P(2,15)*SPP(1) - P(14,15)*SPP(11) + P(15,15)*SPP(3) + P(16,15)*SPP(8));
    nextP(6,8) = P(6,8) + P(1,8)*SF(5) + P(3,8)*SF(4) + P(4,8)*SF(6) - P(2,8)*SPP(1) - P(14,8)*SPP(11) + P(15,8)*SPP(3) + P(16,8)*SPP(8) + dt*(P(6,5) + P(1,5)*SF(5) + P(3,5)*SF(4) + P(4,5)*SF(6) - P(2,5)*SPP(1) - P(14,5)*SPP(11) + P(15,5)*SPP(3) + P(16,5)*SPP(8));
    nextP(6,9) = P(6,9) + P(1,9)*SF(5) + P(3,9)*SF(4) + P(4,9)*SF(6) - P(2,9)*SPP(1) - P(14,9)*SPP(11) + P(15,9)*SPP(3) + P(16,9)*SPP(8) + dt*(P(6,6) + P(1,6)*SF(5) + P(3,6)*SF(4) + P(4,6)*SF(6) - P(2,6)*SPP(1) - P(14,6)*SPP(11) + P(15,6)*SPP(3) + P(16,6)*SPP(8));
    nextP(6,10) = P(6,10) + P(1,10)*SF(5) + P(3,10)*SF(4) + P(4,10)*SF(6) - P(2,10)*SPP(1) - P(14,10)*SPP(11) + P(15,10)*SPP(3) + P(16,10)*SPP(8) + dt*(P(6,7) + P(1,7)*SF(5) + P(3,7)*SF(4) + P(4,7)*SF(6) - P(2,7)*SPP(1) - P(14,7)*SPP(11) + P(15,7)*SPP(3) + P(16,7)*SPP(8));
    nextP(6,11) = P(6,11) + P(1,11)*SF(5) + P(3,11)*SF(4) + P(4,11)*SF(6) - P(2,11)*SPP(1) - P(14,11)*SPP(11) + P(15,11)*SPP(3) + P(16,11)*SPP(8);
    nextP(6,12) = P(6,12) + P(1,12)*SF(5) + P(3,12)*SF(4) + P(4,12)*SF(6) - P(2,12)*SPP(1) - P(14,12)*SPP(11) + P(15,12)*SPP(3) + P(16,12)*SPP(8);
    nextP(6,13) = P(6,13) + P(1,13)*SF(5) + P(3,13)*SF(4) + P(4,13)*SF(6) - P(2,13)*SPP(1) - P(14,13)*SPP(11) + P(15,13)*SPP(3) + P(16,13)*SPP(8);
    nextP(6,14) = P(6,14) + P(1,14)*SF(5) + P(3,14)*SF(4) + P(4,14)*SF(6) - P(2,14)*SPP(1) - P(14,14)*SPP(11) + P(15,14)*SPP(3) + P(16,14)*SPP(8);
    nextP(6,15) = P(6,15) + P(1,15)*SF(5) + P(3,15)*SF(4) + P(4,15)*SF(6) - P(2,15)*SPP(1) - P(14,15)*SPP(11) + P(15,15)*SPP(3) + P(16,15)*SPP(8);
    nextP(6,16) = P(6,16) + P(1,16)*SF(5) + P(3,16)*SF(4) + P(4,16)*SF(6) - P(2,16)*SPP(1) - P(14,16)*SPP(11) + P(15,16)*SPP(3) + P(16,16)*SPP(8);
    nextP(6,17) = P(6,17) + P(1,17)*SF(5) + P(3,17)*SF(4) + P(4,17)*SF(6) - P(2,17)*SPP(1) - P(14,17)*SPP(11) + P(15,17)*SPP(3) + P(16,17)*SPP(8);
    nextP(6,18) = P(6,18) + P(1,18)*SF(5) + P(3,18)*SF(4) + P(4,18)*SF(6) - P(2,18)*SPP(1) - P(14,18)*SPP(11) + P(15,18)*SPP(3) + P(16,18)*SPP(8);
    nextP(6,19) = P(6,19) + P(1,19)*SF(5) + P(3,19)*SF(4) + P(4,19)*SF(6) - P(2,19)*SPP(1) - P(14,19)*SPP(11) + P(15,19)*SPP(3) + P(16,19)*SPP(8);
    nextP(6,20) = P(6,20) + P(1,20)*SF(5) + P(3,20)*SF(4) + P(4,20)*SF(6) - P(2,20)*SPP(1) - P(14,20)*SPP(11) + P(15,20)*SPP(3) + P(16,20)*SPP(8);
    nextP(6,21) = P(6,21) + P(1,21)*SF(5) + P(3,21)*SF(4) + P(4,21)*SF(6) - P(2,21)*SPP(1) - P(14,21)*SPP(11) + P(15,21)*SPP(3) + P(16,21)*SPP(8);
    nextP(6,22) = P(6,22) + P(1,22)*SF(5) + P(3,22)*SF(4) + P(4,22)*SF(6) - P(2,22)*SPP(1) - P(14,22)*SPP(11) + P(15,22)*SPP(3) + P(16,22)*SPP(8);
    nextP(6,23) = P(6,23) + P(1,23)*SF(5) + P(3,23)*SF(4) + P(4,23)*SF(6) - P(2,23)*SPP(1) - P(14,23)*SPP(11) + P(15,23)*SPP(3) + P(16,23)*SPP(8);
    nextP(6,24) = P(6,24) + P(1,24)*SF(5) + P(3,24)*SF(4) + P(4,24)*SF(6) - P(2,24)*SPP(1) - P(14,24)*SPP(11) + P(15,24)*SPP(3) + P(16,24)*SPP(8);
    nextP(7,1) = P(7,1) + P(2,1)*SF(5) + P(4,1)*SF(4) + P(1,1)*SPP(1) - P(3,1)*SPP(5) + P(14,1)*SPP(7) - P(15,1)*SPP(10) - P(16,1)*SPP(2) + SF(10)*(P(7,2) + P(2,2)*SF(5) + P(4,2)*SF(4) + P(1,2)*SPP(1) - P(3,2)*SPP(5) + P(14,2)*SPP(7) - P(15,2)*SPP(10) - P(16,2)*SPP(2)) + SF(12)*(P(7,3) + P(2,3)*SF(5) + P(4,3)*SF(4) + P(1,3)*SPP(1) - P(3,3)*SPP(5) + P(14,3)*SPP(7) - P(15,3)*SPP(10) - P(16,3)*SPP(2)) + SF(11)*(P(7,4) + P(2,4)*SF(5) + P(4,4)*SF(4) + P(1,4)*SPP(1) - P(3,4)*SPP(5) + P(14,4)*SPP(7) - P(15,4)*SPP(10) - P(16,4)*SPP(2)) + SF(15)*(P(7,11) + P(2,11)*SF(5) + P(4,11)*SF(4) + P(1,11)*SPP(1) - P(3,11)*SPP(5) + P(14,11)*SPP(7) - P(15,11)*SPP(10) - P(16,11)*SPP(2)) + SF(16)*(P(7,12) + P(2,12)*SF(5) + P(4,12)*SF(4) + P(1,12)*SPP(1) - P(3,12)*SPP(5) + P(14,12)*SPP(7) - P(15,12)*SPP(10) - P(16,12)*SPP(2)) + SPP(13)*(P(7,13) + P(2,13)*SF(5) + P(4,13)*SF(4) + P(1,13)*SPP(1) - P(3,13)*SPP(5) + P(14,13)*SPP(7) - P(15,13)*SPP(10) - P(16,13)*SPP(2));
    nextP(7,2) = P(7,2) + P(2,2)*SF(5) + P(4,2)*SF(4) + P(1,2)*SPP(1) - P(3,2)*SPP(5) + P(14,2)*SPP(7) - P(15,2)*SPP(10) - P(16,2)*SPP(2) + SF(9)*(P(7,1) + P(2,1)*SF(5) + P(4,1)*SF(4) + P(1,1)*SPP(1) - P(3,1)*SPP(5) + P(14,1)*SPP(7) - P(15,1)*SPP(10) - P(16,1)*SPP(2)) + SF(8)*(P(7,3) + P(2,3)*SF(5) + P(4,3)*SF(4) + P(1,3)*SPP(1) - P(3,3)*SPP(5) + P(14,3)*SPP(7) - P(15,3)*SPP(10) - P(16,3)*SPP(2)) + SF(12)*(P(7,4) + P(2,4)*SF(5) + P(4,4)*SF(4) + P(1,4)*SPP(1) - P(3,4)*SPP(5) + P(14,4)*SPP(7) - P(15,4)*SPP(10) - P(16,4)*SPP(2)) - SF(16)*(P(7,13) + P(2,13)*SF(5) + P(4,13)*SF(4) + P(1,13)*SPP(1) - P(3,13)*SPP(5) + P(14,13)*SPP(7) - P(15,13)*SPP(10) - P(16,13)*SPP(2)) + SPP(13)*(P(7,12) + P(2,12)*SF(5) + P(4,12)*SF(4) + P(1,12)*SPP(1) - P(3,12)*SPP(5) + P(14,12)*SPP(7) - P(15,12)*SPP(10) - P(16,12)*SPP(2)) - (q0*(P(7,11) + P(2,11)*SF(5) + P(4,11)*SF(4) + P(1,11)*SPP(1) - P(3,11)*SPP(5) + P(14,11)*SPP(7) - P(15,11)*SPP(10) - P(16,11)*SPP(2)))/2;
    nextP(7,3) = P(7,3) + P(2,3)*SF(5) + P(4,3)*SF(4) + P(1,3)*SPP(1) - P(3,3)*SPP(5) + P(14,3)*SPP(7) - P(15,3)*SPP(10) - P(16,3)*SPP(2) + SF(7)*(P(7,1) + P(2,1)*SF(5) + P(4,1)*SF(4) + P(1,1)*SPP(1) - P(3,1)*SPP(5) + P(14,1)*SPP(7) - P(15,1)*SPP(10) - P(16,1)*SPP(2)) + SF(11)*(P(7,2) + P(2,2)*SF(5) + P(4,2)*SF(4) + P(1,2)*SPP(1) - P(3,2)*SPP(5) + P(14,2)*SPP(7) - P(15,2)*SPP(10) - P(16,2)*SPP(2)) + SF(9)*(P(7,4) + P(2,4)*SF(5) + P(4,4)*SF(4) + P(1,4)*SPP(1) - P(3,4)*SPP(5) + P(14,4)*SPP(7) - P(15,4)*SPP(10) - P(16,4)*SPP(2)) + SF(15)*(P(7,13) + P(2,13)*SF(5) + P(4,13)*SF(4) + P(1,13)*SPP(1) - P(3,13)*SPP(5) + P(14,13)*SPP(7) - P(15,13)*SPP(10) - P(16,13)*SPP(2)) - SPP(13)*(P(7,11) + P(2,11)*SF(5) + P(4,11)*SF(4) + P(1,11)*SPP(1) - P(3,11)*SPP(5) + P(14,11)*SPP(7) - P(15,11)*SPP(10) - P(16,11)*SPP(2)) - (q0*(P(7,12) + P(2,12)*SF(5) + P(4,12)*SF(4) + P(1,12)*SPP(1) - P(3,12)*SPP(5) + P(14,12)*SPP(7) - P(15,12)*SPP(10) - P(16,12)*SPP(2)))/2;
    nextP(7,4) = P(7,4) + P(2,4)*SF(5) + P(4,4)*SF(4) + P(1,4)*SPP(1) - P(3,4)*SPP(5) + P(14,4)*SPP(7) - P(15,4)*SPP(10) - P(16,4)*SPP(2) + SF(8)*(P(7,1) + P(2,1)*SF(5) + P(4,1)*SF(4) + P(1,1)*SPP(1) - P(3,1)*SPP(5) + P(14,1)*SPP(7) - P(15,1)*SPP(10) - P(16,1)*SPP(2)) + SF(7)*(P(7,2) + P(2,2)*SF(5) + P(4,2)*SF(4) + P(1,2)*SPP(1) - P(3,2)*SPP(5) + P(14,2)*SPP(7) - P(15,2)*SPP(10) - P(16,2)*SPP(2)) + SF(10)*(P(7,3) + P(2,3)*SF(5) + P(4,3)*SF(4) + P(1,3)*SPP(1) - P(3,3)*SPP(5) + P(14,3)*SPP(7) - P(15,3)*SPP(10) - P(16,3)*SPP(2)) + SF(16)*(P(7,11) + P(2,11)*SF(5) + P(4,11)*SF(4) + P(1,11)*SPP(1) - P(3,11)*SPP(5) + P(14,11)*SPP(7) - P(15,11)*SPP(10) - P(16,11)*SPP(2)) - SF(15)*(P(7,12) + P(2,12)*SF(5) + P(4,12)*SF(4) + P(1,12)*SPP(1) - P(3,12)*SPP(5) + P(14,12)*SPP(7) - P(15,12)*SPP(10) - P(16,12)*SPP(2)) - (q0*(P(7,13) + P(2,13)*SF(5) + P(4,13)*SF(4) + P(1,13)*SPP(1) - P(3,13)*SPP(5) + P(14,13)*SPP(7) - P(15,13)*SPP(10) - P(16,13)*SPP(2)))/2;
    nextP(7,5) = P(7,5) + SQ(2) + P(2,5)*SF(5) + P(4,5)*SF(4) + P(1,5)*SPP(1) - P(3,5)*SPP(5) + P(14,5)*SPP(7) - P(15,5)*SPP(10) - P(16,5)*SPP(2) + SF(6)*(P(7,1) + P(2,1)*SF(5) + P(4,1)*SF(4) + P(1,1)*SPP(1) - P(3,1)*SPP(5) + P(14,1)*SPP(7) - P(15,1)*SPP(10) - P(16,1)*SPP(2)) + SF(4)*(P(7,2) + P(2,2)*SF(5) + P(4,2)*SF(4) + P(1,2)*SPP(1) - P(3,2)*SPP(5) + P(14,2)*SPP(7) - P(15,2)*SPP(10) - P(16,2)*SPP(2)) + SPP(1)*(P(7,3) + P(2,3)*SF(5) + P(4,3)*SF(4) + P(1,3)*SPP(1) - P(3,3)*SPP(5) + P(14,3)*SPP(7) - P(15,3)*SPP(10) - P(16,3)*SPP(2)) - SPP(6)*(P(7,4) + P(2,4)*SF(5) + P(4,4)*SF(4) + P(1,4)*SPP(1) - P(3,4)*SPP(5) + P(14,4)*SPP(7) - P(15,4)*SPP(10) - P(16,4)*SPP(2)) + SPP(4)*(P(7,14) + P(2,14)*SF(5) + P(4,14)*SF(4) + P(1,14)*SPP(1) - P(3,14)*SPP(5) + P(14,14)*SPP(7) - P(15,14)*SPP(10) - P(16,14)*SPP(2)) + SPP(9)*(P(7,15) + P(2,15)*SF(5) + P(4,15)*SF(4) + P(1,15)*SPP(1) - P(3,15)*SPP(5) + P(14,15)*SPP(7) - P(15,15)*SPP(10) - P(16,15)*SPP(2)) - SPP(12)*(P(7,16) + P(2,16)*SF(5) + P(4,16)*SF(4) + P(1,16)*SPP(1) - P(3,16)*SPP(5) + P(14,16)*SPP(7) - P(15,16)*SPP(10) - P(16,16)*SPP(2));
    nextP(7,6) = P(7,6) + SQ(1) + P(2,6)*SF(5) + P(4,6)*SF(4) + P(1,6)*SPP(1) - P(3,6)*SPP(5) + P(14,6)*SPP(7) - P(15,6)*SPP(10) - P(16,6)*SPP(2) + SF(5)*(P(7,1) + P(2,1)*SF(5) + P(4,1)*SF(4) + P(1,1)*SPP(1) - P(3,1)*SPP(5) + P(14,1)*SPP(7) - P(15,1)*SPP(10) - P(16,1)*SPP(2)) + SF(4)*(P(7,3) + P(2,3)*SF(5) + P(4,3)*SF(4) + P(1,3)*SPP(1) - P(3,3)*SPP(5) + P(14,3)*SPP(7) - P(15,3)*SPP(10) - P(16,3)*SPP(2)) + SF(6)*(P(7,4) + P(2,4)*SF(5) + P(4,4)*SF(4) + P(1,4)*SPP(1) - P(3,4)*SPP(5) + P(14,4)*SPP(7) - P(15,4)*SPP(10) - P(16,4)*SPP(2)) - SPP(1)*(P(7,2) + P(2,2)*SF(5) + P(4,2)*SF(4) + P(1,2)*SPP(1) - P(3,2)*SPP(5) + P(14,2)*SPP(7) - P(15,2)*SPP(10) - P(16,2)*SPP(2)) + SPP(3)*(P(7,15) + P(2,15)*SF(5) + P(4,15)*SF(4) + P(1,15)*SPP(1) - P(3,15)*SPP(5) + P(14,15)*SPP(7) - P(15,15)*SPP(10) - P(16,15)*SPP(2)) - SPP(11)*(P(7,14) + P(2,14)*SF(5) + P(4,14)*SF(4) + P(1,14)*SPP(1) - P(3,14)*SPP(5) + P(14,14)*SPP(7) - P(15,14)*SPP(10) - P(16,14)*SPP(2)) + SPP(8)*(P(7,16) + P(2,16)*SF(5) + P(4,16)*SF(4) + P(1,16)*SPP(1) - P(3,16)*SPP(5) + P(14,16)*SPP(7) - P(15,16)*SPP(10) - P(16,16)*SPP(2));
    nextP(7,7) = P(7,7) + P(2,7)*SF(5) + P(4,7)*SF(4) + P(1,7)*SPP(1) - P(3,7)*SPP(5) + P(14,7)*SPP(7) - P(15,7)*SPP(10) - P(16,7)*SPP(2) + dvxCov*(SG(7) - 2*q0*q2)^2 + dvyCov*(SG(6) + 2*q0*q1)^2 + SF(5)*(P(7,2) + P(2,2)*SF(5) + P(4,2)*SF(4) + P(1,2)*SPP(1) - P(3,2)*SPP(5) + P(14,2)*SPP(7) - P(15,2)*SPP(10) - P(16,2)*SPP(2)) + SF(4)*(P(7,4) + P(2,4)*SF(5) + P(4,4)*SF(4) + P(1,4)*SPP(1) - P(3,4)*SPP(5) + P(14,4)*SPP(7) - P(15,4)*SPP(10) - P(16,4)*SPP(2)) + SPP(1)*(P(7,1) + P(2,1)*SF(5) + P(4,1)*SF(4) + P(1,1)*SPP(1) - P(3,1)*SPP(5) + P(14,1)*SPP(7) - P(15,1)*SPP(10) - P(16,1)*SPP(2)) - SPP(5)*(P(7,3) + P(2,3)*SF(5) + P(4,3)*SF(4) + P(1,3)*SPP(1) - P(3,3)*SPP(5) + P(14,3)*SPP(7) - P(15,3)*SPP(10) - P(16,3)*SPP(2)) + SPP(7)*(P(7,14) + P(2,14)*SF(5) + P(4,14)*SF(4) + P(1,14)*SPP(1) - P(3,14)*SPP(5) + P(14,14)*SPP(7) - P(15,14)*SPP(10) - P(16,14)*SPP(2)) - SPP(2)*(P(7,16) + P(2,16)*SF(5) + P(4,16)*SF(4) + P(1,16)*SPP(1) - P(3,16)*SPP(5) + P(14,16)*SPP(7) - P(15,16)*SPP(10) - P(16,16)*SPP(2)) - SPP(10)*(P(7,15) + P(2,15)*SF(5) + P(4,15)*SF(4) + P(1,15)*SPP(1) - P(3,15)*SPP(5) + P(14,15)*SPP(7) - P(15,15)*SPP(10) - P(16,15)*SPP(2)) + dvzCov*(SG(2) - SG(3) - SG(4) + SG(5))^2;
    nextP(7,8) = P(7,8) + P(2,8)*SF(5) + P(4,8)*SF(4) + P(1,8)*SPP(1) - P(3,8)*SPP(5) + P(14,8)*SPP(7) - P(15,8)*SPP(10) - P(16,8)*SPP(2) + dt*(P(7,5) + P(2,5)*SF(5) + P(4,5)*SF(4) + P(1,5)*SPP(1) - P(3,5)*SPP(5) + P(14,5)*SPP(7) - P(15,5)*SPP(10) - P(16,5)*SPP(2));
    nextP(7,9) = P(7,9) + P(2,9)*SF(5) + P(4,9)*SF(4) + P(1,9)*SPP(1) - P(3,9)*SPP(5) + P(14,9)*SPP(7) - P(15,9)*SPP(10) - P(16,9)*SPP(2) + dt*(P(7,6) + P(2,6)*SF(5) + P(4,6)*SF(4) + P(1,6)*SPP(1) - P(3,6)*SPP(5) + P(14,6)*SPP(7) - P(15,6)*SPP(10) - P(16,6)*SPP(2));
    nextP(7,10) = P(7,10) + P(2,10)*SF(5) + P(4,10)*SF(4) + P(1,10)*SPP(1) - P(3,10)*SPP(5) + P(14,10)*SPP(7) - P(15,10)*SPP(10) - P(16,10)*SPP(2) + dt*(P(7,7) + P(2,7)*SF(5) + P(4,7)*SF(4) + P(1,7)*SPP(1) - P(3,7)*SPP(5) + P(14,7)*SPP(7) - P(15,7)*SPP(10) - P(16,7)*SPP(2));
    nextP(7,11) = P(7,11) + P(2,11)*SF(5) + P(4,11)*SF(4) + P(1,11)*SPP(1) - P(3,11)*SPP(5) + P(14,11)*SPP(7) - P(15,11)*SPP(10) - P(16,11)*SPP(2);
    nextP(7,12) = P(7,12) + P(2,12)*SF(5) + P(4,12)*SF(4) + P(1,12)*SPP(1) - P(3,12)*SPP(5) + P(14,12)*SPP(7) - P(15,12)*SPP(10) - P(16,12)*SPP(2);
    nextP(7,13) = P(7,13) + P(2,13)*SF(5) + P(4,13)*SF(4) + P(1,13)*SPP(1) - P(3,13)*SPP(5) + P(14,13)*SPP(7) - P(15,13)*SPP(10) - P(16,13)*SPP(2);
    nextP(7,14) = P(7,14) + P(2,14)*SF(5) + P(4,14)*SF(4) + P(1,14)*SPP(1) - P(3,14)*SPP(5) + P(14,14)*SPP(7) - P(15,14)*SPP(10) - P(16,14)*SPP(2);
    nextP(7,15) = P(7,15) + P(2,15)*SF(5) + P(4,15)*SF(4) + P(1,15)*SPP(1) - P(3,15)*SPP(5) + P(14,15)*SPP(7) - P(15,15)*SPP(10) - P(16,15)*SPP(2);
    nextP(7,16) = P(7,16) + P(2,16)*SF(5) + P(4,16)*SF(4) + P(1,16)*SPP(1) - P(3,16)*SPP(5) + P(14,16)*SPP(7) - P(15,16)*SPP(10) - P(16,16)*SPP(2);
    nextP(7,17) = P(7,17) + P(2,17)*SF(5) + P(4,17)*SF(4) + P(1,17)*SPP(1) - P(3,17)*SPP(5) + P(14,17)*SPP(7) - P(15,17)*SPP(10) - P(16,17)*SPP(2);
    nextP(7,18) = P(7,18) + P(2,18)*SF(5) + P(4,18)*SF(4) + P(1,18)*SPP(1) - P(3,18)*SPP(5) + P(14,18)*SPP(7) - P(15,18)*SPP(10) - P(16,18)*SPP(2);
    nextP(7,19) = P(7,19) + P(2,19)*SF(5) + P(4,19)*SF(4) + P(1,19)*SPP(1) - P(3,19)*SPP(5) + P(14,19)*SPP(7) - P(15,19)*SPP(10) - P(16,19)*SPP(2);
    nextP(7,20) = P(7,20) + P(2,20)*SF(5) + P(4,20)*SF(4) + P(1,20)*SPP(1) - P(3,20)*SPP(5) + P(14,20)*SPP(7) - P(15,20)*SPP(10) - P(16,20)*SPP(2);
    nextP(7,21) = P(7,21) + P(2,21)*SF(5) + P(4,21)*SF(4) + P(1,21)*SPP(1) - P(3,21)*SPP(5) + P(14,21)*SPP(7) - P(15,21)*SPP(10) - P(16,21)*SPP(2);
    nextP(7,22) = P(7,22) + P(2,22)*SF(5) + P(4,22)*SF(4) + P(1,22)*SPP(1) - P(3,22)*SPP(5) + P(14,22)*SPP(7) - P(15,22)*SPP(10) - P(16,22)*SPP(2);
    nextP(7,23) = P(7,23) + P(2,23)*SF(5) + P(4,23)*SF(4) + P(1,23)*SPP(1) - P(3,23)*SPP(5) + P(14,23)*SPP(7) - P(15,23)*SPP(10) - P(16,23)*SPP(2);
    nextP(7,24) = P(7,24) + P(2,24)*SF(5) + P(4,24)*SF(4) + P(1,24)*SPP(1) - P(3,24)*SPP(5) + P(14,24)*SPP(7) - P(15,24)*SPP(10) - P(16,24)*SPP(2);
    nextP(8,1) = P(8,1) + P(5,1)*dt + SF(10)*(P(8,2) + P(5,2)*dt) + SF(12)*(P(8,3) + P(5,3)*dt) + SF(11)*(P(8,4) + P(5,4)*dt) + SF(15)*(P(8,11) + P(5,11)*dt) + SF(16)*(P(8,12) + P(5,12)*dt) + SPP(13)*(P(8,13) + P(5,13)*dt);
    nextP(8,2) = P(8,2) + P(5,2)*dt + SF(9)*(P(8,1) + P(5,1)*dt) + SF(8)*(P(8,3) + P(5,3)*dt) + SF(12)*(P(8,4) + P(5,4)*dt) - SF(16)*(P(8,13) + P(5,13)*dt) + SPP(13)*(P(8,12) + P(5,12)*dt) - (q0*(P(8,11) + P(5,11)*dt))/2;
    nextP(8,3) = P(8,3) + P(5,3)*dt + SF(7)*(P(8,1) + P(5,1)*dt) + SF(11)*(P(8,2) + P(5,2)*dt) + SF(9)*(P(8,4) + P(5,4)*dt) + SF(15)*(P(8,13) + P(5,13)*dt) - SPP(13)*(P(8,11) + P(5,11)*dt) - (q0*(P(8,12) + P(5,12)*dt))/2;
    nextP(8,4) = P(8,4) + P(5,4)*dt + SF(8)*(P(8,1) + P(5,1)*dt) + SF(7)*(P(8,2) + P(5,2)*dt) + SF(10)*(P(8,3) + P(5,3)*dt) + SF(16)*(P(8,11) + P(5,11)*dt) - SF(15)*(P(8,12) + P(5,12)*dt) - (q0*(P(8,13) + P(5,13)*dt))/2;
    nextP(8,5) = P(8,5) + P(5,5)*dt + SF(4)*(P(8,2) + P(5,2)*dt) + SF(6)*(P(8,1) + P(5,1)*dt) + SPP(1)*(P(8,3) + P(5,3)*dt) - SPP(6)*(P(8,4) + P(5,4)*dt) + SPP(4)*(P(8,14) + P(5,14)*dt) + SPP(9)*(P(8,15) + P(5,15)*dt) - SPP(12)*(P(8,16) + P(5,16)*dt);
    nextP(8,6) = P(8,6) + P(5,6)*dt + SF(5)*(P(8,1) + P(5,1)*dt) + SF(4)*(P(8,3) + P(5,3)*dt) + SF(6)*(P(8,4) + P(5,4)*dt) - SPP(1)*(P(8,2) + P(5,2)*dt) + SPP(3)*(P(8,15) + P(5,15)*dt) - SPP(11)*(P(8,14) + P(5,14)*dt) + SPP(8)*(P(8,16) + P(5,16)*dt);
    nextP(8,7) = P(8,7) + P(5,7)*dt + SF(5)*(P(8,2) + P(5,2)*dt) + SF(4)*(P(8,4) + P(5,4)*dt) + SPP(1)*(P(8,1) + P(5,1)*dt) - SPP(5)*(P(8,3) + P(5,3)*dt) - SPP(2)*(P(8,16) + P(5,16)*dt) + SPP(7)*(P(8,14) + P(5,14)*dt) - SPP(10)*(P(8,15) + P(5,15)*dt);
    nextP(8,8) = P(8,8) + P(5,8)*dt + dt*(P(8,5) + P(5,5)*dt);
    nextP(8,9) = P(8,9) + P(5,9)*dt + dt*(P(8,6) + P(5,6)*dt);
    nextP(8,10) = P(8,10) + P(5,10)*dt + dt*(P(8,7) + P(5,7)*dt);
    nextP(8,11) = P(8,11) + P(5,11)*dt;
    nextP(8,12) = P(8,12) + P(5,12)*dt;
    nextP(8,13) = P(8,13) + P(5,13)*dt;
    nextP(8,14) = P(8,14) + P(5,14)*dt;
    nextP(8,15) = P(8,15) + P(5,15)*dt;
    nextP(8,16) = P(8,16) + P(5,16)*dt;
    nextP(8,17) = P(8,17) + P(5,17)*dt;
    nextP(8,18) = P(8,18) + P(5,18)*dt;
    nextP(8,19) = P(8,19) + P(5,19)*dt;
    nextP(8,20) = P(8,20) + P(5,20)*dt;
    nextP(8,21) = P(8,21) + P(5,21)*dt;
    nextP(8,22) = P(8,22) + P(5,22)*dt;
    nextP(8,23) = P(8,23) + P(5,23)*dt;
    nextP(8,24) = P(8,24) + P(5,24)*dt;
    nextP(9,1) = P(9,1) + P(6,1)*dt + SF(10)*(P(9,2) + P(6,2)*dt) + SF(12)*(P(9,3) + P(6,3)*dt) + SF(11)*(P(9,4) + P(6,4)*dt) + SF(15)*(P(9,11) + P(6,11)*dt) + SF(16)*(P(9,12) + P(6,12)*dt) + SPP(13)*(P(9,13) + P(6,13)*dt);
    nextP(9,2) = P(9,2) + P(6,2)*dt + SF(9)*(P(9,1) + P(6,1)*dt) + SF(8)*(P(9,3) + P(6,3)*dt) + SF(12)*(P(9,4) + P(6,4)*dt) - SF(16)*(P(9,13) + P(6,13)*dt) + SPP(13)*(P(9,12) + P(6,12)*dt) - (q0*(P(9,11) + P(6,11)*dt))/2;
    nextP(9,3) = P(9,3) + P(6,3)*dt + SF(7)*(P(9,1) + P(6,1)*dt) + SF(11)*(P(9,2) + P(6,2)*dt) + SF(9)*(P(9,4) + P(6,4)*dt) + SF(15)*(P(9,13) + P(6,13)*dt) - SPP(13)*(P(9,11) + P(6,11)*dt) - (q0*(P(9,12) + P(6,12)*dt))/2;
    nextP(9,4) = P(9,4) + P(6,4)*dt + SF(8)*(P(9,1) + P(6,1)*dt) + SF(7)*(P(9,2) + P(6,2)*dt) + SF(10)*(P(9,3) + P(6,3)*dt) + SF(16)*(P(9,11) + P(6,11)*dt) - SF(15)*(P(9,12) + P(6,12)*dt) - (q0*(P(9,13) + P(6,13)*dt))/2;
    nextP(9,5) = P(9,5) + P(6,5)*dt + SF(4)*(P(9,2) + P(6,2)*dt) + SF(6)*(P(9,1) + P(6,1)*dt) + SPP(1)*(P(9,3) + P(6,3)*dt) - SPP(6)*(P(9,4) + P(6,4)*dt) + SPP(4)*(P(9,14) + P(6,14)*dt) + SPP(9)*(P(9,15) + P(6,15)*dt) - SPP(12)*(P(9,16) + P(6,16)*dt);
    nextP(9,6) = P(9,6) + P(6,6)*dt + SF(5)*(P(9,1) + P(6,1)*dt) + SF(4)*(P(9,3) + P(6,3)*dt) + SF(6)*(P(9,4) + P(6,4)*dt) - SPP(1)*(P(9,2) + P(6,2)*dt) + SPP(3)*(P(9,15) + P(6,15)*dt) - SPP(11)*(P(9,14) + P(6,14)*dt) + SPP(8)*(P(9,16) + P(6,16)*dt);
    nextP(9,7) = P(9,7) + P(6,7)*dt + SF(5)*(P(9,2) + P(6,2)*dt) + SF(4)*(P(9,4) + P(6,4)*dt) + SPP(1)*(P(9,1) + P(6,1)*dt) - SPP(5)*(P(9,3) + P(6,3)*dt) - SPP(2)*(P(9,16) + P(6,16)*dt) + SPP(7)*(P(9,14) + P(6,14)*dt) - SPP(10)*(P(9,15) + P(6,15)*dt);
    nextP(9,8) = P(9,8) + P(6,8)*dt + dt*(P(9,5) + P(6,5)*dt);
    nextP(9,9) = P(9,9) + P(6,9)*dt + dt*(P(9,6) + P(6,6)*dt);
    nextP(9,10) = P(9,10) + P(6,10)*dt + dt*(P(9,7) + P(6,7)*dt);
    nextP(9,11) = P(9,11) + P(6,11)*dt;
    nextP(9,12) = P(9,12) + P(6,12)*dt;
    nextP(9,13) = P(9,13) + P(6,13)*dt;
    nextP(9,14) = P(9,14) + P(6,14)*dt;
    nextP(9,15) = P(9,15) + P(6,15)*dt;
    nextP(9,16) = P(9,16) + P(6,16)*dt;
    nextP(9,17) = P(9,17) + P(6,17)*dt;
    nextP(9,18) = P(9,18) + P(6,18)*dt;
    nextP(9,19) = P(9,19) + P(6,19)*dt;
    nextP(9,20) = P(9,20) + P(6,20)*dt;
    nextP(9,21) = P(9,21) + P(6,21)*dt;
    nextP(9,22) = P(9,22) + P(6,22)*dt;
    nextP(9,23) = P(9,23) + P(6,23)*dt;
    nextP(9,24) = P(9,24) + P(6,24)*dt;
    nextP(10,1) = P(10,1) + P(7,1)*dt + SF(10)*(P(10,2) + P(7,2)*dt) + SF(12)*(P(10,3) + P(7,3)*dt) + SF(11)*(P(10,4) + P(7,4)*dt) + SF(15)*(P(10,11) + P(7,11)*dt) + SF(16)*(P(10,12) + P(7,12)*dt) + SPP(13)*(P(10,13) + P(7,13)*dt);
    nextP(10,2) = P(10,2) + P(7,2)*dt + SF(9)*(P(10,1) + P(7,1)*dt) + SF(8)*(P(10,3) + P(7,3)*dt) + SF(12)*(P(10,4) + P(7,4)*dt) - SF(16)*(P(10,13) + P(7,13)*dt) + SPP(13)*(P(10,12) + P(7,12)*dt) - (q0*(P(10,11) + P(7,11)*dt))/2;
    nextP(10,3) = P(10,3) + P(7,3)*dt + SF(7)*(P(10,1) + P(7,1)*dt) + SF(11)*(P(10,2) + P(7,2)*dt) + SF(9)*(P(10,4) + P(7,4)*dt) + SF(15)*(P(10,13) + P(7,13)*dt) - SPP(13)*(P(10,11) + P(7,11)*dt) - (q0*(P(10,12) + P(7,12)*dt))/2;
    nextP(10,4) = P(10,4) + P(7,4)*dt + SF(8)*(P(10,1) + P(7,1)*dt) + SF(7)*(P(10,2) + P(7,2)*dt) + SF(10)*(P(10,3) + P(7,3)*dt) + SF(16)*(P(10,11) + P(7,11)*dt) - SF(15)*(P(10,12) + P(7,12)*dt) - (q0*(P(10,13) + P(7,13)*dt))/2;
    nextP(10,5) = P(10,5) + P(7,5)*dt + SF(4)*(P(10,2) + P(7,2)*dt) + SF(6)*(P(10,1) + P(7,1)*dt) + SPP(1)*(P(10,3) + P(7,3)*dt) - SPP(6)*(P(10,4) + P(7,4)*dt) + SPP(4)*(P(10,14) + P(7,14)*dt) + SPP(9)*(P(10,15) + P(7,15)*dt) - SPP(12)*(P(10,16) + P(7,16)*dt);
    nextP(10,6) = P(10,6) + P(7,6)*dt + SF(5)*(P(10,1) + P(7,1)*dt) + SF(4)*(P(10,3) + P(7,3)*dt) + SF(6)*(P(10,4) + P(7,4)*dt) - SPP(1)*(P(10,2) + P(7,2)*dt) + SPP(3)*(P(10,15) + P(7,15)*dt) - SPP(11)*(P(10,14) + P(7,14)*dt) + SPP(8)*(P(10,16) + P(7,16)*dt);
    nextP(10,7) = P(10,7) + P(7,7)*dt + SF(5)*(P(10,2) + P(7,2)*dt) + SF(4)*(P(10,4) + P(7,4)*dt) + SPP(1)*(P(10,1) + P(7,1)*dt) - SPP(5)*(P(10,3) + P(7,3)*dt) - SPP(2)*(P(10,16) + P(7,16)*dt) + SPP(7)*(P(10,14) + P(7,14)*dt) - SPP(10)*(P(10,15) + P(7,15)*dt);
    nextP(10,8) = P(10,8) + P(7,8)*dt + dt*(P(10,5) + P(7,5)*dt);
    nextP(10,9) = P(10,9) + P(7,9)*dt + dt*(P(10,6) + P(7,6)*dt);
    nextP(10,10) = P(10,10) + P(7,10)*dt + dt*(P(10,7) + P(7,7)*dt);
    nextP(10,11) = P(10,11) + P(7,11)*dt;
    nextP(10,12) = P(10,12) + P(7,12)*dt;
    nextP(10,13) = P(10,13) + P(7,13)*dt;
    nextP(10,14) = P(10,14) + P(7,14)*dt;
    nextP(10,15) = P(10,15) + P(7,15)*dt;
    nextP(10,16) = P(10,16) + P(7,16)*dt;
    nextP(10,17) = P(10,17) + P(7,17)*dt;
    nextP(10,18) = P(10,18) + P(7,18)*dt;
    nextP(10,19) = P(10,19) + P(7,19)*dt;
    nextP(10,20) = P(10,20) + P(7,20)*dt;
    nextP(10,21) = P(10,21) + P(7,21)*dt;
    nextP(10,22) = P(10,22) + P(7,22)*dt;
    nextP(10,23) = P(10,23) + P(7,23)*dt;
    nextP(10,24) = P(10,24) + P(7,24)*dt;
    nextP(11,1) = P(11,1) + P(11,2)*SF(10) + P(11,3)*SF(12) + P(11,4)*SF(11) + P(11,11)*SF(15) + P(11,12)*SF(16) + P(11,13)*SPP(13);
    nextP(11,2) = P(11,2) + P(11,1)*SF(9) + P(11,3)*SF(8) + P(11,4)*SF(12) - P(11,13)*SF(16) + P(11,12)*SPP(13) - (P(11,11)*q0)/2;
    nextP(11,3) = P(11,3) + P(11,1)*SF(7) + P(11,2)*SF(11) + P(11,4)*SF(9) + P(11,13)*SF(15) - P(11,11)*SPP(13) - (P(11,12)*q0)/2;
    nextP(11,4) = P(11,4) + P(11,1)*SF(8) + P(11,2)*SF(7) + P(11,3)*SF(10) + P(11,11)*SF(16) - P(11,12)*SF(15) - (P(11,13)*q0)/2;
    nextP(11,5) = P(11,5) + P(11,2)*SF(4) + P(11,1)*SF(6) + P(11,3)*SPP(1) - P(11,4)*SPP(6) + P(11,14)*SPP(4) + P(11,15)*SPP(9) - P(11,16)*SPP(12);
    nextP(11,6) = P(11,6) + P(11,1)*SF(5) + P(11,3)*SF(4) + P(11,4)*SF(6) - P(11,2)*SPP(1) + P(11,15)*SPP(3) + P(11,16)*SPP(8) - P(11,14)*SPP(11);
    nextP(11,7) = P(11,7) + P(11,2)*SF(5) + P(11,4)*SF(4) + P(11,1)*SPP(1) - P(11,3)*SPP(5) - P(11,16)*SPP(2) + P(11,14)*SPP(7) - P(11,15)*SPP(10);
    nextP(11,8) = P(11,8) + P(11,5)*dt;
    nextP(11,9) = P(11,9) + P(11,6)*dt;
    nextP(11,10) = P(11,10) + P(11,7)*dt;
    nextP(11,11) = P(11,11);
    nextP(11,12) = P(11,12);
    nextP(11,13) = P(11,13);
    nextP(11,14) = P(11,14);
    nextP(11,15) = P(11,15);
    nextP(11,16) = P(11,16);
    nextP(11,17) = P(11,17);
    nextP(11,18) = P(11,18);
    nextP(11,19) = P(11,19);
    nextP(11,20) = P(11,20);
    nextP(11,21) = P(11,21);
    nextP(11,22) = P(11,22);
    nextP(11,23) = P(11,23);
    nextP(11,24) = P(11,24);
    nextP(12,1) = P(12,1) + P(12,2)*SF(10) + P(12,3)*SF(12) + P(12,4)*SF(11) + P(12,11)*SF(15) + P(12,12)*SF(16) + P(12,13)*SPP(13);
    nextP(12,2) = P(12,2) + P(12,1)*SF(9) + P(12,3)*SF(8) + P(12,4)*SF(12) - P(12,13)*SF(16) + P(12,12)*SPP(13) - (P(12,11)*q0)/2;
    nextP(12,3) = P(12,3) + P(12,1)*SF(7) + P(12,2)*SF(11) + P(12,4)*SF(9) + P(12,13)*SF(15) - P(12,11)*SPP(13) - (P(12,12)*q0)/2;
    nextP(12,4) = P(12,4) + P(12,1)*SF(8) + P(12,2)*SF(7) + P(12,3)*SF(10) + P(12,11)*SF(16) - P(12,12)*SF(15) - (P(12,13)*q0)/2;
    nextP(12,5) = P(12,5) + P(12,2)*SF(4) + P(12,1)*SF(6) + P(12,3)*SPP(1) - P(12,4)*SPP(6) + P(12,14)*SPP(4) + P(12,15)*SPP(9) - P(12,16)*SPP(12);
    nextP(12,6) = P(12,6) + P(12,1)*SF(5) + P(12,3)*SF(4) + P(12,4)*SF(6) - P(12,2)*SPP(1) + P(12,15)*SPP(3) + P(12,16)*SPP(8) - P(12,14)*SPP(11);
    nextP(12,7) = P(12,7) + P(12,2)*SF(5) + P(12,4)*SF(4) + P(12,1)*SPP(1) - P(12,3)*SPP(5) - P(12,16)*SPP(2) + P(12,14)*SPP(7) - P(12,15)*SPP(10);
    nextP(12,8) = P(12,8) + P(12,5)*dt;
    nextP(12,9) = P(12,9) + P(12,6)*dt;
    nextP(12,10) = P(12,10) + P(12,7)*dt;
    nextP(12,11) = P(12,11);
    nextP(12,12) = P(12,12);
    nextP(12,13) = P(12,13);
    nextP(12,14) = P(12,14);
    nextP(12,15) = P(12,15);
    nextP(12,16) = P(12,16);
    nextP(12,17) = P(12,17);
    nextP(12,18) = P(12,18);
    nextP(12,19) = P(12,19);
    nextP(12,20) = P(12,20);
    nextP(12,21) = P(12,21);
    nextP(12,22) = P(12,22);
    nextP(12,23) = P(12,23);
    nextP(12,24) = P(12,24);
    nextP(13,1) = P(13,1) + P(13,2)*SF(10) + P(13,3)*SF(12) + P(13,4)*SF(11) + P(13,11)*SF(15) + P(13,12)*SF(16) + P(13,13)*SPP(13);
    nextP(13,2) = P(13,2) + P(13,1)*SF(9) + P(13,3)*SF(8) + P(13,4)*SF(12) - P(13,13)*SF(16) + P(13,12)*SPP(13) - (P(13,11)*q0)/2;
    nextP(13,3) = P(13,3) + P(13,1)*SF(7) + P(13,2)*SF(11) + P(13,4)*SF(9) + P(13,13)*SF(15) - P(13,11)*SPP(13) - (P(13,12)*q0)/2;
    nextP(13,4) = P(13,4) + P(13,1)*SF(8) + P(13,2)*SF(7) + P(13,3)*SF(10) + P(13,11)*SF(16) - P(13,12)*SF(15) - (P(13,13)*q0)/2;
    nextP(13,5) = P(13,5) + P(13,2)*SF(4) + P(13,1)*SF(6) + P(13,3)*SPP(1) - P(13,4)*SPP(6) + P(13,14)*SPP(4) + P(13,15)*SPP(9) - P(13,16)*SPP(12);
    nextP(13,6) = P(13,6) + P(13,1)*SF(5) + P(13,3)*SF(4) + P(13,4)*SF(6) - P(13,2)*SPP(1) + P(13,15)*SPP(3) + P(13,16)*SPP(8) - P(13,14)*SPP(11);
    nextP(13,7) = P(13,7) + P(13,2)*SF(5) + P(13,4)*SF(4) + P(13,1)*SPP(1) - P(13,3)*SPP(5) - P(13,16)*SPP(2) + P(13,14)*SPP(7) - P(13,15)*SPP(10);
    nextP(13,8) = P(13,8) + P(13,5)*dt;
    nextP(13,9) = P(13,9) + P(13,6)*dt;
    nextP(13,10) = P(13,10) + P(13,7)*dt;
    nextP(13,11) = P(13,11);
    nextP(13,12) = P(13,12);
    nextP(13,13) = P(13,13);
    nextP(13,14) = P(13,14);
    nextP(13,15) = P(13,15);
    nextP(13,16) = P(13,16);
    nextP(13,17) = P(13,17);
    nextP(13,18) = P(13,18);
    nextP(13,19) = P(13,19);
    nextP(13,20) = P(13,20);
    nextP(13,21) = P(13,21);
    nextP(13,22) = P(13,22);
    nextP(13,23) = P(13,23);
    nextP(13,24) = P(13,24);
    nextP(14,1) = P(14,1) + P(14,2)*SF(10) + P(14,3)*SF(12) + P(14,4)*SF(11) + P(14,11)*SF(15) + P(14,12)*SF(16) + P(14,13)*SPP(13);
    nextP(14,2) = P(14,2) + P(14,1)*SF(9) + P(14,3)*SF(8) + P(14,4)*SF(12) - P(14,13)*SF(16) + P(14,12)*SPP(13) - (P(14,11)*q0)/2;
    nextP(14,3) = P(14,3) + P(14,1)*SF(7) + P(14,2)*SF(11) + P(14,4)*SF(9) + P(14,13)*SF(15) - P(14,11)*SPP(13) - (P(14,12)*q0)/2;
    nextP(14,4) = P(14,4) + P(14,1)*SF(8) + P(14,2)*SF(7) + P(14,3)*SF(10) + P(14,11)*SF(16) - P(14,12)*SF(15) - (P(14,13)*q0)/2;
    nextP(14,5) = P(14,5) + P(14,2)*SF(4) + P(14,1)*SF(6) + P(14,3)*SPP(1) - P(14,4)*SPP(6) + P(14,14)*SPP(4) + P(14,15)*SPP(9) - P(14,16)*SPP(12);
    nextP(14,6) = P(14,6) + P(14,1)*SF(5) + P(14,3)*SF(4) + P(14,4)*SF(6) - P(14,2)*SPP(1) + P(14,15)*SPP(3) + P(14,16)*SPP(8) - P(14,14)*SPP(11);
    nextP(14,7) = P(14,7) + P(14,2)*SF(5) + P(14,4)*SF(4) + P(14,1)*SPP(1) - P(14,3)*SPP(5) - P(14,16)*SPP(2) + P(14,14)*SPP(7) - P(14,15)*SPP(10);
    nextP(14,8) = P(14,8) + P(14,5)*dt;
    nextP(14,9) = P(14,9) + P(14,6)*dt;
    nextP(14,10) = P(14,10) + P(14,7)*dt;
    nextP(14,11) = P(14,11);
    nextP(14,12) = P(14,12);
    nextP(14,13) = P(14,13);
    nextP(14,14) = P(14,14);
    nextP(14,15) = P(14,15);
    nextP(14,16) = P(14,16);
    nextP(14,17) = P(14,17);
    nextP(14,18) = P(14,18);
    nextP(14,19) = P(14,19);
    nextP(14,20) = P(14,20);
    nextP(14,21) = P(14,21);
    nextP(14,22) = P(14,22);
    nextP(14,23) = P(14,23);
    nextP(14,24) = P(14,24);
    nextP(15,1) = P(15,1) + P(15,2)*SF(10) + P(15,3)*SF(12) + P(15,4)*SF(11) + P(15,11)*SF(15) + P(15,12)*SF(16) + P(15,13)*SPP(13);
    nextP(15,2) = P(15,2) + P(15,1)*SF(9) + P(15,3)*SF(8) + P(15,4)*SF(12) - P(15,13)*SF(16) + P(15,12)*SPP(13) - (P(15,11)*q0)/2;
    nextP(15,3) = P(15,3) + P(15,1)*SF(7) + P(15,2)*SF(11) + P(15,4)*SF(9) + P(15,13)*SF(15) - P(15,11)*SPP(13) - (P(15,12)*q0)/2;
    nextP(15,4) = P(15,4) + P(15,1)*SF(8) + P(15,2)*SF(7) + P(15,3)*SF(10) + P(15,11)*SF(16) - P(15,12)*SF(15) - (P(15,13)*q0)/2;
    nextP(15,5) = P(15,5) + P(15,2)*SF(4) + P(15,1)*SF(6) + P(15,3)*SPP(1) - P(15,4)*SPP(6) + P(15,14)*SPP(4) + P(15,15)*SPP(9) - P(15,16)*SPP(12);
    nextP(15,6) = P(15,6) + P(15,1)*SF(5) + P(15,3)*SF(4) + P(15,4)*SF(6) - P(15,2)*SPP(1) + P(15,15)*SPP(3) + P(15,16)*SPP(8) - P(15,14)*SPP(11);
    nextP(15,7) = P(15,7) + P(15,2)*SF(5) + P(15,4)*SF(4) + P(15,1)*SPP(1) - P(15,3)*SPP(5) - P(15,16)*SPP(2) + P(15,14)*SPP(7) - P(15,15)*SPP(10);
    nextP(15,8) = P(15,8) + P(15,5)*dt;
    nextP(15,9) = P(15,9) + P(15,6)*dt;
    nextP(15,10) = P(15,10) + P(15,7)*dt;
    nextP(15,11) = P(15,11);
    nextP(15,12) = P(15,12);
    nextP(15,13) = P(15,13);
    nextP(15,14) = P(15,14);
    nextP(15,15) = P(15,15);
    nextP(15,16) = P(15,16);
    nextP(15,17) = P(15,17);
    nextP(15,18) = P(15,18);
    nextP(15,19) = P(15,19);
    nextP(15,20) = P(15,20);
    nextP(15,21) = P(15,21);
    nextP(15,22) = P(15,22);
    nextP(15,23) = P(15,23);
    nextP(15,24) = P(15,24);
    nextP(16,1) = P(16,1) + P(16,2)*SF(10) + P(16,3)*SF(12) + P(16,4)*SF(11) + P(16,11)*SF(15) + P(16,12)*SF(16) + P(16,13)*SPP(13);
    nextP(16,2) = P(16,2) + P(16,1)*SF(9) + P(16,3)*SF(8) + P(16,4)*SF(12) - P(16,13)*SF(16) + P(16,12)*SPP(13) - (P(16,11)*q0)/2;
    nextP(16,3) = P(16,3) + P(16,1)*SF(7) + P(16,2)*SF(11) + P(16,4)*SF(9) + P(16,13)*SF(15) - P(16,11)*SPP(13) - (P(16,12)*q0)/2;
    nextP(16,4) = P(16,4) + P(16,1)*SF(8) + P(16,2)*SF(7) + P(16,3)*SF(10) + P(16,11)*SF(16) - P(16,12)*SF(15) - (P(16,13)*q0)/2;
    nextP(16,5) = P(16,5) + P(16,2)*SF(4) + P(16,1)*SF(6) + P(16,3)*SPP(1) - P(16,4)*SPP(6) + P(16,14)*SPP(4) + P(16,15)*SPP(9) - P(16,16)*SPP(12);
    nextP(16,6) = P(16,6) + P(16,1)*SF(5) + P(16,3)*SF(4) + P(16,4)*SF(6) - P(16,2)*SPP(1) + P(16,15)*SPP(3) + P(16,16)*SPP(8) - P(16,14)*SPP(11);
    nextP(16,7) = P(16,7) + P(16,2)*SF(5) + P(16,4)*SF(4) + P(16,1)*SPP(1) - P(16,3)*SPP(5) - P(16,16)*SPP(2) + P(16,14)*SPP(7) - P(16,15)*SPP(10);
    nextP(16,8) = P(16,8) + P(16,5)*dt;
    nextP(16,9) = P(16,9) + P(16,6)*dt;
    nextP(16,10) = P(16,10) + P(16,7)*dt;
    nextP(16,11) = P(16,11);
    nextP(16,12) = P(16,12);
    nextP(16,13) = P(16,13);
    nextP(16,14) = P(16,14);
    nextP(16,15) = P(16,15);
    nextP(16,16) = P(16,16);
    nextP(16,17) = P(16,17);
    nextP(16,18) = P(16,18);
    nextP(16,19) = P(16,19);
    nextP(16,20) = P(16,20);
    nextP(16,21) = P(16,21);
    nextP(16,22) = P(16,22);
    nextP(16,23) = P(16,23);
    nextP(16,24) = P(16,24);
    nextP(17,1) = P(17,1) + P(17,2)*SF(10) + P(17,3)*SF(12) + P(17,4)*SF(11) + P(17,11)*SF(15) + P(17,12)*SF(16) + P(17,13)*SPP(13);
    nextP(17,2) = P(17,2) + P(17,1)*SF(9) + P(17,3)*SF(8) + P(17,4)*SF(12) - P(17,13)*SF(16) + P(17,12)*SPP(13) - (P(17,11)*q0)/2;
    nextP(17,3) = P(17,3) + P(17,1)*SF(7) + P(17,2)*SF(11) + P(17,4)*SF(9) + P(17,13)*SF(15) - P(17,11)*SPP(13) - (P(17,12)*q0)/2;
    nextP(17,4) = P(17,4) + P(17,1)*SF(8) + P(17,2)*SF(7) + P(17,3)*SF(10) + P(17,11)*SF(16) - P(17,12)*SF(15) - (P(17,13)*q0)/2;
    nextP(17,5) = P(17,5) + P(17,2)*SF(4) + P(17,1)*SF(6) + P(17,3)*SPP(1) - P(17,4)*SPP(6) + P(17,14)*SPP(4) + P(17,15)*SPP(9) - P(17,16)*SPP(12);
    nextP(17,6) = P(17,6) + P(17,1)*SF(5) + P(17,3)*SF(4) + P(17,4)*SF(6) - P(17,2)*SPP(1) + P(17,15)*SPP(3) + P(17,16)*SPP(8) - P(17,14)*SPP(11);
    nextP(17,7) = P(17,7) + P(17,2)*SF(5) + P(17,4)*SF(4) + P(17,1)*SPP(1) - P(17,3)*SPP(5) - P(17,16)*SPP(2) + P(17,14)*SPP(7) - P(17,15)*SPP(10);
    nextP(17,8) = P(17,8) + P(17,5)*dt;
    nextP(17,9) = P(17,9) + P(17,6)*dt;
    nextP(17,10) = P(17,10) + P(17,7)*dt;
    nextP(17,11) = P(17,11);
    nextP(17,12) = P(17,12);
    nextP(17,13) = P(17,13);
    nextP(17,14) = P(17,14);
    nextP(17,15) = P(17,15);
    nextP(17,16) = P(17,16);
    nextP(17,17) = P(17,17);
    nextP(17,18) = P(17,18);
    nextP(17,19) = P(17,19);
    nextP(17,20) = P(17,20);
    nextP(17,21) = P(17,21);
    nextP(17,22) = P(17,22);
    nextP(17,23) = P(17,23);
    nextP(17,24) = P(17,24);
    nextP(18,1) = P(18,1) + P(18,2)*SF(10) + P(18,3)*SF(12) + P(18,4)*SF(11) + P(18,11)*SF(15) + P(18,12)*SF(16) + P(18,13)*SPP(13);
    nextP(18,2) = P(18,2) + P(18,1)*SF(9) + P(18,3)*SF(8) + P(18,4)*SF(12) - P(18,13)*SF(16) + P(18,12)*SPP(13) - (P(18,11)*q0)/2;
    nextP(18,3) = P(18,3) + P(18,1)*SF(7) + P(18,2)*SF(11) + P(18,4)*SF(9) + P(18,13)*SF(15) - P(18,11)*SPP(13) - (P(18,12)*q0)/2;
    nextP(18,4) = P(18,4) + P(18,1)*SF(8) + P(18,2)*SF(7) + P(18,3)*SF(10) + P(18,11)*SF(16) - P(18,12)*SF(15) - (P(18,13)*q0)/2;
    nextP(18,5) = P(18,5) + P(18,2)*SF(4) + P(18,1)*SF(6) + P(18,3)*SPP(1) - P(18,4)*SPP(6) + P(18,14)*SPP(4) + P(18,15)*SPP(9) - P(18,16)*SPP(12);
    nextP(18,6) = P(18,6) + P(18,1)*SF(5) + P(18,3)*SF(4) + P(18,4)*SF(6) - P(18,2)*SPP(1) + P(18,15)*SPP(3) + P(18,16)*SPP(8) - P(18,14)*SPP(11);
    nextP(18,7) = P(18,7) + P(18,2)*SF(5) + P(18,4)*SF(4) + P(18,1)*SPP(1) - P(18,3)*SPP(5) - P(18,16)*SPP(2) + P(18,14)*SPP(7) - P(18,15)*SPP(10);
    nextP(18,8) = P(18,8) + P(18,5)*dt;
    nextP(18,9) = P(18,9) + P(18,6)*dt;
    nextP(18,10) = P(18,10) + P(18,7)*dt;
    nextP(18,11) = P(18,11);
    nextP(18,12) = P(18,12);
    nextP(18,13) = P(18,13);
    nextP(18,14) = P(18,14);
    nextP(18,15) = P(18,15);
    nextP(18,16) = P(18,16);
    nextP(18,17) = P(18,17);
    nextP(18,18) = P(18,18);
    nextP(18,19) = P(18,19);
    nextP(18,20) = P(18,20);
    nextP(18,21) = P(18,21);
    nextP(18,22) = P(18,22);
    nextP(18,23) = P(18,23);
    nextP(18,24) = P(18,24);
    nextP(19,1) = P(19,1) + P(19,2)*SF(10) + P(19,3)*SF(12) + P(19,4)*SF(11) + P(19,11)*SF(15) + P(19,12)*SF(16) + P(19,13)*SPP(13);
    nextP(19,2) = P(19,2) + P(19,1)*SF(9) + P(19,3)*SF(8) + P(19,4)*SF(12) - P(19,13)*SF(16) + P(19,12)*SPP(13) - (P(19,11)*q0)/2;
    nextP(19,3) = P(19,3) + P(19,1)*SF(7) + P(19,2)*SF(11) + P(19,4)*SF(9) + P(19,13)*SF(15) - P(19,11)*SPP(13) - (P(19,12)*q0)/2;
    nextP(19,4) = P(19,4) + P(19,1)*SF(8) + P(19,2)*SF(7) + P(19,3)*SF(10) + P(19,11)*SF(16) - P(19,12)*SF(15) - (P(19,13)*q0)/2;
    nextP(19,5) = P(19,5) + P(19,2)*SF(4) + P(19,1)*SF(6) + P(19,3)*SPP(1) - P(19,4)*SPP(6) + P(19,14)*SPP(4) + P(19,15)*SPP(9) - P(19,16)*SPP(12);
    nextP(19,6) = P(19,6) + P(19,1)*SF(5) + P(19,3)*SF(4) + P(19,4)*SF(6) - P(19,2)*SPP(1) + P(19,15)*SPP(3) + P(19,16)*SPP(8) - P(19,14)*SPP(11);
    nextP(19,7) = P(19,7) + P(19,2)*SF(5) + P(19,4)*SF(4) + P(19,1)*SPP(1) - P(19,3)*SPP(5) - P(19,16)*SPP(2) + P(19,14)*SPP(7) - P(19,15)*SPP(10);
    nextP(19,8) = P(19,8) + P(19,5)*dt;
    nextP(19,9) = P(19,9) + P(19,6)*dt;
    nextP(19,10) = P(19,10) + P(19,7)*dt;
    nextP(19,11) = P(19,11);
    nextP(19,12) = P(19,12);
    nextP(19,13) = P(19,13);
    nextP(19,14) = P(19,14);
    nextP(19,15) = P(19,15);
    nextP(19,16) = P(19,16);
    nextP(19,17) = P(19,17);
    nextP(19,18) = P(19,18);
    nextP(19,19) = P(19,19);
    nextP(19,20) = P(19,20);
    nextP(19,21) = P(19,21);
    nextP(19,22) = P(19,22);
    nextP(19,23) = P(19,23);
    nextP(19,24) = P(19,24);
    nextP(20,1) = P(20,1) + P(20,2)*SF(10) + P(20,3)*SF(12) + P(20,4)*SF(11) + P(20,11)*SF(15) + P(20,12)*SF(16) + P(20,13)*SPP(13);
    nextP(20,2) = P(20,2) + P(20,1)*SF(9) + P(20,3)*SF(8) + P(20,4)*SF(12) - P(20,13)*SF(16) + P(20,12)*SPP(13) - (P(20,11)*q0)/2;
    nextP(20,3) = P(20,3) + P(20,1)*SF(7) + P(20,2)*SF(11) + P(20,4)*SF(9) + P(20,13)*SF(15) - P(20,11)*SPP(13) - (P(20,12)*q0)/2;
    nextP(20,4) = P(20,4) + P(20,1)*SF(8) + P(20,2)*SF(7) + P(20,3)*SF(10) + P(20,11)*SF(16) - P(20,12)*SF(15) - (P(20,13)*q0)/2;
    nextP(20,5) = P(20,5) + P(20,2)*SF(4) + P(20,1)*SF(6) + P(20,3)*SPP(1) - P(20,4)*SPP(6) + P(20,14)*SPP(4) + P(20,15)*SPP(9) - P(20,16)*SPP(12);
    nextP(20,6) = P(20,6) + P(20,1)*SF(5) + P(20,3)*SF(4) + P(20,4)*SF(6) - P(20,2)*SPP(1) + P(20,15)*SPP(3) + P(20,16)*SPP(8) - P(20,14)*SPP(11);
    nextP(20,7) = P(20,7) + P(20,2)*SF(5) + P(20,4)*SF(4) + P(20,1)*SPP(1) - P(20,3)*SPP(5) - P(20,16)*SPP(2) + P(20,14)*SPP(7) - P(20,15)*SPP(10);
    nextP(20,8) = P(20,8) + P(20,5)*dt;
    nextP(20,9) = P(20,9) + P(20,6)*dt;
    nextP(20,10) = P(20,10) + P(20,7)*dt;
    nextP(20,11) = P(20,11);
    nextP(20,12) = P(20,12);
    nextP(20,13) = P(20,13);
    nextP(20,14) = P(20,14);
    nextP(20,15) = P(20,15);
    nextP(20,16) = P(20,16);
    nextP(20,17) = P(20,17);
    nextP(20,18) = P(20,18);
    nextP(20,19) = P(20,19);
    nextP(20,20) = P(20,20);
    nextP(20,21) = P(20,21);
    nextP(20,22) = P(20,22);
    nextP(20,23) = P(20,23);
    nextP(20,24) = P(20,24);
    nextP(21,1) = P(21,1) + P(21,2)*SF(10) + P(21,3)*SF(12) + P(21,4)*SF(11) + P(21,11)*SF(15) + P(21,12)*SF(16) + P(21,13)*SPP(13);
    nextP(21,2) = P(21,2) + P(21,1)*SF(9) + P(21,3)*SF(8) + P(21,4)*SF(12) - P(21,13)*SF(16) + P(21,12)*SPP(13) - (P(21,11)*q0)/2;
    nextP(21,3) = P(21,3) + P(21,1)*SF(7) + P(21,2)*SF(11) + P(21,4)*SF(9) + P(21,13)*SF(15) - P(21,11)*SPP(13) - (P(21,12)*q0)/2;
    nextP(21,4) = P(21,4) + P(21,1)*SF(8) + P(21,2)*SF(7) + P(21,3)*SF(10) + P(21,11)*SF(16) - P(21,12)*SF(15) - (P(21,13)*q0)/2;
    nextP(21,5) = P(21,5) + P(21,2)*SF(4) + P(21,1)*SF(6) + P(21,3)*SPP(1) - P(21,4)*SPP(6) + P(21,14)*SPP(4) + P(21,15)*SPP(9) - P(21,16)*SPP(12);
    nextP(21,6) = P(21,6) + P(21,1)*SF(5) + P(21,3)*SF(4) + P(21,4)*SF(6) - P(21,2)*SPP(1) + P(21,15)*SPP(3) + P(21,16)*SPP(8) - P(21,14)*SPP(11);
    nextP(21,7) = P(21,7) + P(21,2)*SF(5) + P(21,4)*SF(4) + P(21,1)*SPP(1) - P(21,3)*SPP(5) - P(21,16)*SPP(2) + P(21,14)*SPP(7) - P(21,15)*SPP(10);
    nextP(21,8) = P(21,8) + P(21,5)*dt;
    nextP(21,9) = P(21,9) + P(21,6)*dt;
    nextP(21,10) = P(21,10) + P(21,7)*dt;
    nextP(21,11) = P(21,11);
    nextP(21,12) = P(21,12);
    nextP(21,13) = P(21,13);
    nextP(21,14) = P(21,14);
    nextP(21,15) = P(21,15);
    nextP(21,16) = P(21,16);
    nextP(21,17) = P(21,17);
    nextP(21,18) = P(21,18);
    nextP(21,19) = P(21,19);
    nextP(21,20) = P(21,20);
    nextP(21,21) = P(21,21);
    nextP(21,22) = P(21,22);
    nextP(21,23) = P(21,23);
    nextP(21,24) = P(21,24);
    nextP(22,1) = P(22,1) + P(22,2)*SF(10) + P(22,3)*SF(12) + P(22,4)*SF(11) + P(22,11)*SF(15) + P(22,12)*SF(16) + P(22,13)*SPP(13);
    nextP(22,2) = P(22,2) + P(22,1)*SF(9) + P(22,3)*SF(8) + P(22,4)*SF(12) - P(22,13)*SF(16) + P(22,12)*SPP(13) - (P(22,11)*q0)/2;
    nextP(22,3) = P(22,3) + P(22,1)*SF(7) + P(22,2)*SF(11) + P(22,4)*SF(9) + P(22,13)*SF(15) - P(22,11)*SPP(13) - (P(22,12)*q0)/2;
    nextP(22,4) = P(22,4) + P(22,1)*SF(8) + P(22,2)*SF(7) + P(22,3)*SF(10) + P(22,11)*SF(16) - P(22,12)*SF(15) - (P(22,13)*q0)/2;
    nextP(22,5) = P(22,5) + P(22,2)*SF(4) + P(22,1)*SF(6) + P(22,3)*SPP(1) - P(22,4)*SPP(6) + P(22,14)*SPP(4) + P(22,15)*SPP(9) - P(22,16)*SPP(12);
    nextP(22,6) = P(22,6) + P(22,1)*SF(5) + P(22,3)*SF(4) + P(22,4)*SF(6) - P(22,2)*SPP(1) + P(22,15)*SPP(3) + P(22,16)*SPP(8) - P(22,14)*SPP(11);
    nextP(22,7) = P(22,7) + P(22,2)*SF(5) + P(22,4)*SF(4) + P(22,1)*SPP(1) - P(22,3)*SPP(5) - P(22,16)*SPP(2) + P(22,14)*SPP(7) - P(22,15)*SPP(10);
    nextP(22,8) = P(22,8) + P(22,5)*dt;
    nextP(22,9) = P(22,9) + P(22,6)*dt;
    nextP(22,10) = P(22,10) + P(22,7)*dt;
    nextP(22,11) = P(22,11);
    nextP(22,12) = P(22,12);
    nextP(22,13) = P(22,13);
    nextP(22,14) = P(22,14);
    nextP(22,15) = P(22,15);
    nextP(22,16) = P(22,16);
    nextP(22,17) = P(22,17);
    nextP(22,18) = P(22,18);
    nextP(22,19) = P(22,19);
    nextP(22,20) = P(22,20);
    nextP(22,21) = P(22,21);
    nextP(22,22) = P(22,22);
    nextP(22,23) = P(22,23);
    nextP(22,24) = P(22,24);
    nextP(23,1) = P(23,1) + P(23,2)*SF(10) + P(23,3)*SF(12) + P(23,4)*SF(11) + P(23,11)*SF(15) + P(23,12)*SF(16) + P(23,13)*SPP(13);
    nextP(23,2) = P(23,2) + P(23,1)*SF(9) + P(23,3)*SF(8) + P(23,4)*SF(12) - P(23,13)*SF(16) + P(23,12)*SPP(13) - (P(23,11)*q0)/2;
    nextP(23,3) = P(23,3) + P(23,1)*SF(7) + P(23,2)*SF(11) + P(23,4)*SF(9) + P(23,13)*SF(15) - P(23,11)*SPP(13) - (P(23,12)*q0)/2;
    nextP(23,4) = P(23,4) + P(23,1)*SF(8) + P(23,2)*SF(7) + P(23,3)*SF(10) + P(23,11)*SF(16) - P(23,12)*SF(15) - (P(23,13)*q0)/2;
    nextP(23,5) = P(23,5) + P(23,2)*SF(4) + P(23,1)*SF(6) + P(23,3)*SPP(1) - P(23,4)*SPP(6) + P(23,14)*SPP(4) + P(23,15)*SPP(9) - P(23,16)*SPP(12);
    nextP(23,6) = P(23,6) + P(23,1)*SF(5) + P(23,3)*SF(4) + P(23,4)*SF(6) - P(23,2)*SPP(1) + P(23,15)*SPP(3) + P(23,16)*SPP(8) - P(23,14)*SPP(11);
    nextP(23,7) = P(23,7) + P(23,2)*SF(5) + P(23,4)*SF(4) + P(23,1)*SPP(1) - P(23,3)*SPP(5) - P(23,16)*SPP(2) + P(23,14)*SPP(7) - P(23,15)*SPP(10);
    nextP(23,8) = P(23,8) + P(23,5)*dt;
    nextP(23,9) = P(23,9) + P(23,6)*dt;
    nextP(23,10) = P(23,10) + P(23,7)*dt;
    nextP(23,11) = P(23,11);
    nextP(23,12) = P(23,12);
    nextP(23,13) = P(23,13);
    nextP(23,14) = P(23,14);
    nextP(23,15) = P(23,15);
    nextP(23,16) = P(23,16);
    nextP(23,17) = P(23,17);
    nextP(23,18) = P(23,18);
    nextP(23,19) = P(23,19);
    nextP(23,20) = P(23,20);
    nextP(23,21) = P(23,21);
    nextP(23,22) = P(23,22);
    nextP(23,23) = P(23,23);
    nextP(23,24) = P(23,24);
    nextP(24,1) = P(24,1) + P(24,2)*SF(10) + P(24,3)*SF(12) + P(24,4)*SF(11) + P(24,11)*SF(15) + P(24,12)*SF(16) + P(24,13)*SPP(13);
    nextP(24,2) = P(24,2) + P(24,1)*SF(9) + P(24,3)*SF(8) + P(24,4)*SF(12) - P(24,13)*SF(16) + P(24,12)*SPP(13) - (P(24,11)*q0)/2;
    nextP(24,3) = P(24,3) + P(24,1)*SF(7) + P(24,2)*SF(11) + P(24,4)*SF(9) + P(24,13)*SF(15) - P(24,11)*SPP(13) - (P(24,12)*q0)/2;
    nextP(24,4) = P(24,4) + P(24,1)*SF(8) + P(24,2)*SF(7) + P(24,3)*SF(10) + P(24,11)*SF(16) - P(24,12)*SF(15) - (P(24,13)*q0)/2;
    nextP(24,5) = P(24,5) + P(24,2)*SF(4) + P(24,1)*SF(6) + P(24,3)*SPP(1) - P(24,4)*SPP(6) + P(24,14)*SPP(4) + P(24,15)*SPP(9) - P(24,16)*SPP(12);
    nextP(24,6) = P(24,6) + P(24,1)*SF(5) + P(24,3)*SF(4) + P(24,4)*SF(6) - P(24,2)*SPP(1) + P(24,15)*SPP(3) + P(24,16)*SPP(8) - P(24,14)*SPP(11);
    nextP(24,7) = P(24,7) + P(24,2)*SF(5) + P(24,4)*SF(4) + P(24,1)*SPP(1) - P(24,3)*SPP(5) - P(24,16)*SPP(2) + P(24,14)*SPP(7) - P(24,15)*SPP(10);
    nextP(24,8) = P(24,8) + P(24,5)*dt;
    nextP(24,9) = P(24,9) + P(24,6)*dt;
    nextP(24,10) = P(24,10) + P(24,7)*dt;
    nextP(24,11) = P(24,11);
    nextP(24,12) = P(24,12);
    nextP(24,13) = P(24,13);
    nextP(24,14) = P(24,14);
    nextP(24,15) = P(24,15);
    nextP(24,16) = P(24,16);
    nextP(24,17) = P(24,17);
    nextP(24,18) = P(24,18);
    nextP(24,19) = P(24,19);
    nextP(24,20) = P(24,20);
    nextP(24,21) = P(24,21);
    nextP(24,22) = P(24,22);
    nextP(24,23) = P(24,23);
    nextP(24,24) = P(24,24);
    
    % Add the process noise
    for i = 1:24
        nextP(i,i) = nextP(i,i) + processNoise(i);
    end
    
    % If on ground, inhibit accelerometer bias updates by setting the coresponding
    % covariance terms to zero. To be efficient, the corresponding terms should
    % also not be calculated above
    if onGround
        % Inhibit Acc bias state updates and covariance growth
        nextP(14:16,:) = single(0);
        nextP(:,14:16) = single(0);
    end
    
    % If on ground or no magnetometer fitted, inhibit magnetometer bias updates by
    % setting the coresponding covariance terms to zero. To be efficient, the
    % corresponding terms should also not be calculated above
    if onGround || ~useCompass
        % Inhibit magnetic flux state updates and covariance growth
        nextP(19:24,:) = single(0);
        nextP(:,19:24) = single(0);
    end
    
    % If on ground or not using airspeed sensing, inhibit wind velocity
    % covariance growth by setting the coresponding covariance terms to zero.
    % To be % efficient, the corresponding terms should also not be calculated above
    if onGround || ~useAirspeed
        % Inhibit Wind velocity state updates and covariance growth
        nextP(17:18,:) = 0.0;
        nextP(:,17:18) = 0.0;
    end
    
    % If the total position variance exceds 1E6 (1000m), then stop covariance
    % growth by setting the predicted to the previous values
    % This prevent an ill conditioned matrix from occurring for long periods
    % without GPS
    if (P(8,8) + P(9,9)) > 1E6
        nextP(8:9,:) = P(8:9,:);
        nextP(:,8:9) = P(:,8:9);
    end
    
    % Force symmetry on the covariance matrix to prevent ill-conditioning
    % of the matrix which would cause the filter to blow-up
    for i = 2:24
        for j = 1:(i-1)
            temp = 0.5*(nextP(i,j) + nextP(j,i));
            nextP(i,j) = temp;
            nextP(j,i) = temp;
        end
    end
    
    % reset the accumulated values
    storedDelAng = single([0;0;0]);
    storedDelVel = single([0;0;0]);
    dt = single(0.0);
    
else
    nextP = P;
end

end
